simulink model "untitled"  (R2016a)
(part 5 of 5)

      mask Display: e = 0.06;c1 = [120 150 230]/255;c2 = ([120 150 230]+0)/383;c3 = ([120 150 230]+128)/383;patch([0 1 1 0],[0 0 1 1],c1);patch([0 1 1 1-e 1-e 0+e],[0 0 1 1-e 0+e 0+e],c2);patch([0 0 1 1-e 0+e 0+e],[0 1 1 1-e 1-e 0+e],c3);plot([0 1 1 0 0],[0 0 1 1 0]);disp('weights');
  "IW{2,1}(336,:)'" : Constant  Value=[0.57929667385134542;-0.78903803203994949;-0.58353476825563777;0.33313549786967889;0.5285986546184529;0.55820885952562127;-0.15831488004105437;0.041845262259330829;0.26856481467974563;0.19459032736235027]
      mask Display: e = 0.06;c1 = [120 150 230]/255;c2 = ([120 150 230]+0)/383;c3 = ([120 150 230]+128)/383;patch([0 1 1 0],[0 0 1 1],c1);patch([0 1 1 1-e 1-e 0+e],[0 0 1 1-e 0+e 0+e],c2);patch([0 0 1 1-e 0+e 0+e],[0 1 1 1-e 1-e 0+e],c3);plot([0 1 1 0 0],[0 0 1 1 0]);disp('weights');
  "IW{2,1}(337,:)'" : Constant  Value=[0.12574676902065979;0.1437303392596804;-1.0210731034248322;-0.76168646026924314;-0.43069041398995267;-0.42377470805759543;-0.92888594177016837;-0.74632505329387844;0.7159189367543517;0.21230092583291182]
      mask Display: e = 0.06;c1 = [120 150 230]/255;c2 = ([120 150 230]+0)/383;c3 = ([120 150 230]+128)/383;patch([0 1 1 0],[0 0 1 1],c1);patch([0 1 1 1-e 1-e 0+e],[0 0 1 1-e 0+e 0+e],c2);patch([0 0 1 1-e 0+e 0+e],[0 1 1 1-e 1-e 0+e],c3);plot([0 1 1 0 0],[0 0 1 1 0]);disp('weights');
  "IW{2,1}(338,:)'" : Constant  Value=[-0.87962689838467056;-0.81965574813773967;0.28812259044425648;0.6537668743923607;0.64909098817751765;0.61059084148729448;0.26188896114050575;-0.10762086270333238;-0.21705727199956715;0.37912970515334743]
      mask Display: e = 0.06;c1 = [120 150 230]/255;c2 = ([120 150 230]+0)/383;c3 = ([120 150 230]+128)/383;patch([0 1 1 0],[0 0 1 1],c1);patch([0 1 1 1-e 1-e 0+e],[0 0 1 1-e 0+e 0+e],c2);patch([0 0 1 1-e 0+e 0+e],[0 1 1 1-e 1-e 0+e],c3);plot([0 1 1 0 0],[0 0 1 1 0]);disp('weights');
  "IW{2,1}(339,:)'" : Constant  Value=[0.27086385814243769;0.13068510614586601;0.24134099648815127;-0.17928302930622905;0.82971681131724795;0.71135694066192445;-0.40450383589249345;0.42312354405169722;-0.51855680944157401;-0.31572508040730729]
      mask Display: e = 0.06;c1 = [120 150 230]/255;c2 = ([120 150 230]+0)/383;c3 = ([120 150 230]+128)/383;patch([0 1 1 0],[0 0 1 1],c1);patch([0 1 1 1-e 1-e 0+e],[0 0 1 1-e 0+e 0+e],c2);patch([0 0 1 1-e 0+e 0+e],[0 1 1 1-e 1-e 0+e],c3);plot([0 1 1 0 0],[0 0 1 1 0]);disp('weights');
  "IW{2,1}(34,:)'" : Constant  Value=[-0.0557140173148791;-0.47020898151700219;-0.10773546464442435;0.13793814800358678;0.0086097713284211119;0.054232313057208437;-1.3206898062037267;-0.5570232407889194;0.42551871848387929;-0.34291539655271253]
      mask Display: e = 0.06;c1 = [120 150 230]/255;c2 = ([120 150 230]+0)/383;c3 = ([120 150 230]+128)/383;patch([0 1 1 0],[0 0 1 1],c1);patch([0 1 1 1-e 1-e 0+e],[0 0 1 1-e 0+e 0+e],c2);patch([0 0 1 1-e 0+e 0+e],[0 1 1 1-e 1-e 0+e],c3);plot([0 1 1 0 0],[0 0 1 1 0]);disp('weights');
  "IW{2,1}(340,:)'" : Constant  Value=[0.67675704174660012;0.29451796126330321;0.96052544413959351;-0.59395989110112135;0.20754162488392677;0.042921057940714935;-0.63021749818323047;-0.10388797316770837;-0.55730109200499489;-0.8694954715348181]
      mask Display: e = 0.06;c1 = [120 150 230]/255;c2 = ([120 150 230]+0)/383;c3 = ([120 150 230]+128)/383;patch([0 1 1 0],[0 0 1 1],c1);patch([0 1 1 1-e 1-e 0+e],[0 0 1 1-e 0+e 0+e],c2);patch([0 0 1 1-e 0+e 0+e],[0 1 1 1-e 1-e 0+e],c3);plot([0 1 1 0 0],[0 0 1 1 0]);disp('weights');
  "IW{2,1}(341,:)'" : Constant  Value=[0.50441264093641003;-0.25814916788099879;0.5273849263763507;0.070525504378618736;-0.85715718129830487;0.22282102719382685;0.11137503921468966;0.15108209667316697;0.47461080777254527;-1.0033026714827977]
      mask Display: e = 0.06;c1 = [120 150 230]/255;c2 = ([120 150 230]+0)/383;c3 = ([120 150 230]+128)/383;patch([0 1 1 0],[0 0 1 1],c1);patch([0 1 1 1-e 1-e 0+e],[0 0 1 1-e 0+e 0+e],c2);patch([0 0 1 1-e 0+e 0+e],[0 1 1 1-e 1-e 0+e],c3);plot([0 1 1 0 0],[0 0 1 1 0]);disp('weights');
  "IW{2,1}(342,:)'" : Constant  Value=[-0.87120151971974302;-0.21701047633843468;0.22343161213378757;-0.6224636306634812;-0.18118189058358763;0.77302593300289923;0.063648446964245042;-0.33024680040415128;0.61297869563987939;0.62661425915964464]
      mask Display: e = 0.06;c1 = [120 150 230]/255;c2 = ([120 150 230]+0)/383;c3 = ([120 150 230]+128)/383;patch([0 1 1 0],[0 0 1 1],c1);patch([0 1 1 1-e 1-e 0+e],[0 0 1 1-e 0+e 0+e],c2);patch([0 0 1 1-e 0+e 0+e],[0 1 1 1-e 1-e 0+e],c3);plot([0 1 1 0 0],[0 0 1 1 0]);disp('weights');
  "IW{2,1}(343,:)'" : Constant  Value=[0.54778667415285753;0.58942993005933753;-0.82715214046328522;-0.42267861457146078;1.217645261929982;0.41030733543075537;-0.48105634702976574;-0.63559529927366576;0.44469140820414194;0.68942657577069366]
      mask Display: e = 0.06;c1 = [120 150 230]/255;c2 = ([120 150 230]+0)/383;c3 = ([120 150 230]+128)/383;patch([0 1 1 0],[0 0 1 1],c1);patch([0 1 1 1-e 1-e 0+e],[0 0 1 1-e 0+e 0+e],c2);patch([0 0 1 1-e 0+e 0+e],[0 1 1 1-e 1-e 0+e],c3);plot([0 1 1 0 0],[0 0 1 1 0]);disp('weights');
  "IW{2,1}(344,:)'" : Constant  Value=[0.80938005282717895;0.85758702347541127;0.3249857359421256;0.068660961528306613;-0.48979054333668026;0.68731063432055062;0.13924348683501817;0.12645778251410511;0.42804861718142606;0.30521647390760931]
      mask Display: e = 0.06;c1 = [120 150 230]/255;c2 = ([120 150 230]+0)/383;c3 = ([120 150 230]+128)/383;patch([0 1 1 0],[0 0 1 1],c1);patch([0 1 1 1-e 1-e 0+e],[0 0 1 1-e 0+e 0+e],c2);patch([0 0 1 1-e 0+e 0+e],[0 1 1 1-e 1-e 0+e],c3);plot([0 1 1 0 0],[0 0 1 1 0]);disp('weights');
  "IW{2,1}(345,:)'" : Constant  Value=[-0.40642866004188194;0.024144431082813451;-1.0230073088457663;-0.95248385746212494;0.72926259142932381;0.30665424718799306;-0.96967684388735786;-0.20945754302261479;-0.39772236198321215;0.71881238198133679]
      mask Display: e = 0.06;c1 = [120 150 230]/255;c2 = ([120 150 230]+0)/383;c3 = ([120 150 230]+128)/383;patch([0 1 1 0],[0 0 1 1],c1);patch([0 1 1 1-e 1-e 0+e],[0 0 1 1-e 0+e 0+e],c2);patch([0 0 1 1-e 0+e 0+e],[0 1 1 1-e 1-e 0+e],c3);plot([0 1 1 0 0],[0 0 1 1 0]);disp('weights');
  "IW{2,1}(346,:)'" : Constant  Value=[1.3740864718913919;0.22871612043931461;-0.044941575484340718;0.6616130294723428;-0.2189939835849456;0.57109137173194335;-0.48540204603619996;0.37566365540689645;-0.52135066902196248;0.10168152866206817]
      mask Display: e = 0.06;c1 = [120 150 230]/255;c2 = ([120 150 230]+0)/383;c3 = ([120 150 230]+128)/383;patch([0 1 1 0],[0 0 1 1],c1);patch([0 1 1 1-e 1-e 0+e],[0 0 1 1-e 0+e 0+e],c2);patch([0 0 1 1-e 0+e 0+e],[0 1 1 1-e 1-e 0+e],c3);plot([0 1 1 0 0],[0 0 1 1 0]);disp('weights');
  "IW{2,1}(347,:)'" : Constant  Value=[0.29248266901944847;-0.33621530376745251;-0.036164134244412352;-0.014456472781074908;-0.29890516910801945;-0.0024103397765527501;-1.0913384164665245;-0.58722890720668386;0.20481619829248193;0.040425924896277027]
      mask Display: e = 0.06;c1 = [120 150 230]/255;c2 = ([120 150 230]+0)/383;c3 = ([120 150 230]+128)/383;patch([0 1 1 0],[0 0 1 1],c1);patch([0 1 1 1-e 1-e 0+e],[0 0 1 1-e 0+e 0+e],c2);patch([0 0 1 1-e 0+e 0+e],[0 1 1 1-e 1-e 0+e],c3);plot([0 1 1 0 0],[0 0 1 1 0]);disp('weights');
  "IW{2,1}(348,:)'" : Constant  Value=[0.066871656522572154;-0.82037360738171827;-1.1829225017254741;-0.11652694921625323;0.4760845225460491;-0.24870797400433475;-0.33779280137749595;-0.3870624604689627;1.1401042150744649;-0.12733608401848256]
      mask Display: e = 0.06;c1 = [120 150 230]/255;c2 = ([120 150 230]+0)/383;c3 = ([120 150 230]+128)/383;patch([0 1 1 0],[0 0 1 1],c1);patch([0 1 1 1-e 1-e 0+e],[0 0 1 1-e 0+e 0+e],c2);patch([0 0 1 1-e 0+e 0+e],[0 1 1 1-e 1-e 0+e],c3);plot([0 1 1 0 0],[0 0 1 1 0]);disp('weights');
  "IW{2,1}(349,:)'" : Constant  Value=[-0.56516748165346065;0.60421432434592071;0.21477667628823882;-0.37962152691604534;0.054230828961916944;0.97713641951169294;0.34032689677335731;-0.22209678073966532;0.69491764586228777;0.40837973620708379]
      mask Display: e = 0.06;c1 = [120 150 230]/255;c2 = ([120 150 230]+0)/383;c3 = ([120 150 230]+128)/383;patch([0 1 1 0],[0 0 1 1],c1);patch([0 1 1 1-e 1-e 0+e],[0 0 1 1-e 0+e 0+e],c2);patch([0 0 1 1-e 0+e 0+e],[0 1 1 1-e 1-e 0+e],c3);plot([0 1 1 0 0],[0 0 1 1 0]);disp('weights');
  "IW{2,1}(35,:)'" : Constant  Value=[-0.25760074676464095;-0.28380985445048007;0.43164066332849033;0.23220168279956635;0.56055874690034724;0.81979353327154014;0.072753955941441018;-0.014426558695554342;-0.071318431922984982;-0.47703848064843912]
      mask Display: e = 0.06;c1 = [120 150 230]/255;c2 = ([120 150 230]+0)/383;c3 = ([120 150 230]+128)/383;patch([0 1 1 0],[0 0 1 1],c1);patch([0 1 1 1-e 1-e 0+e],[0 0 1 1-e 0+e 0+e],c2);patch([0 0 1 1-e 0+e 0+e],[0 1 1 1-e 1-e 0+e],c3);plot([0 1 1 0 0],[0 0 1 1 0]);disp('weights');
  "IW{2,1}(350,:)'" : Constant  Value=[0.051988509795972401;-0.013574912572032562;-0.28560378849152268;-0.32799987653965129;1.3044047508544199;0.43736308271531554;0.071266929416620328;0.73520543165915775;0.10884565625748632;0.25695621700303634]
      mask Display: e = 0.06;c1 = [120 150 230]/255;c2 = ([120 150 230]+0)/383;c3 = ([120 150 230]+128)/383;patch([0 1 1 0],[0 0 1 1],c1);patch([0 1 1 1-e 1-e 0+e],[0 0 1 1-e 0+e 0+e],c2);patch([0 0 1 1-e 0+e 0+e],[0 1 1 1-e 1-e 0+e],c3);plot([0 1 1 0 0],[0 0 1 1 0]);disp('weights');
  "IW{2,1}(351,:)'" : Constant  Value=[0.4568469818767768;0.33566359392055301;0.5049775876308441;-1.1445276549307513;-0.062160417784633715;0.36349307929056063;0.056913164235412275;0.10142049361460195;0.83007833319535318;-0.92565819038237251]
      mask Display: e = 0.06;c1 = [120 150 230]/255;c2 = ([120 150 230]+0)/383;c3 = ([120 150 230]+128)/383;patch([0 1 1 0],[0 0 1 1],c1);patch([0 1 1 1-e 1-e 0+e],[0 0 1 1-e 0+e 0+e],c2);patch([0 0 1 1-e 0+e 0+e],[0 1 1 1-e 1-e 0+e],c3);plot([0 1 1 0 0],[0 0 1 1 0]);disp('weights');
  "IW{2,1}(352,:)'" : Constant  Value=[-0.88703160304489614;-0.95132318021638718;-0.071861533145697376;-0.42033187199910793;-0.68579336170567229;0.35422349162839978;-0.20304709238721164;-0.13214983308353762;0.47337758454097267;0.15078308159578074]
      mask Display: e = 0.06;c1 = [120 150 230]/255;c2 = ([120 150 230]+0)/383;c3 = ([120 150 230]+128)/383;patch([0 1 1 0],[0 0 1 1],c1);patch([0 1 1 1-e 1-e 0+e],[0 0 1 1-e 0+e 0+e],c2);patch([0 0 1 1-e 0+e 0+e],[0 1 1 1-e 1-e 0+e],c3);plot([0 1 1 0 0],[0 0 1 1 0]);disp('weights');
  "IW{2,1}(353,:)'" : Constant  Value=[0.53782537655597384;-1.0045125582834515;0.30134495879826806;0.54230596767481742;-0.11476579937739612;-0.31631782729707281;-0.49763177218689092;0.47994082141207151;-0.026801952215077307;0.25824481163233315]
      mask Display: e = 0.06;c1 = [120 150 230]/255;c2 = ([120 150 230]+0)/383;c3 = ([120 150 230]+128)/383;patch([0 1 1 0],[0 0 1 1],c1);patch([0 1 1 1-e 1-e 0+e],[0 0 1 1-e 0+e 0+e],c2);patch([0 0 1 1-e 0+e 0+e],[0 1 1 1-e 1-e 0+e],c3);plot([0 1 1 0 0],[0 0 1 1 0]);disp('weights');
  "IW{2,1}(354,:)'" : Constant  Value=[-0.41358424712483965;-0.4329293804487403;-0.029573647317088669;-1.2035042893054049;-0.52506569755795507;-0.090459746021540999;-0.83104269463153191;-0.56242756805362537;0.80415249041968218;-0.76295105731743029]
      mask Display: e = 0.06;c1 = [120 150 230]/255;c2 = ([120 150 230]+0)/383;c3 = ([120 150 230]+128)/383;patch([0 1 1 0],[0 0 1 1],c1);patch([0 1 1 1-e 1-e 0+e],[0 0 1 1-e 0+e 0+e],c2);patch([0 0 1 1-e 0+e 0+e],[0 1 1 1-e 1-e 0+e],c3);plot([0 1 1 0 0],[0 0 1 1 0]);disp('weights');
  "IW{2,1}(355,:)'" : Constant  Value=[0.26135712427590718;0.32178024612794087;-0.2015877707363507;-0.56893396997562329;0.85311359616962334;0.77329604180705036;0.18423955850823046;-0.22726419478735588;1.0460001041156679;-1.1010704916311156]
      mask Display: e = 0.06;c1 = [120 150 230]/255;c2 = ([120 150 230]+0)/383;c3 = ([120 150 230]+128)/383;patch([0 1 1 0],[0 0 1 1],c1);patch([0 1 1 1-e 1-e 0+e],[0 0 1 1-e 0+e 0+e],c2);patch([0 0 1 1-e 0+e 0+e],[0 1 1 1-e 1-e 0+e],c3);plot([0 1 1 0 0],[0 0 1 1 0]);disp('weights');
  "IW{2,1}(356,:)'" : Constant  Value=[0.12593724696620373;-0.88317548884339514;0.61782360547129;0.3650623555503672;0.84964646887594097;-0.060897734797931147;-0.09226266712536807;0.95533325883592723;0.21782434532452424;-0.5450519926170927]
      mask Display: e = 0.06;c1 = [120 150 230]/255;c2 = ([120 150 230]+0)/383;c3 = ([120 150 230]+128)/383;patch([0 1 1 0],[0 0 1 1],c1);patch([0 1 1 1-e 1-e 0+e],[0 0 1 1-e 0+e 0+e],c2);patch([0 0 1 1-e 0+e 0+e],[0 1 1 1-e 1-e 0+e],c3);plot([0 1 1 0 0],[0 0 1 1 0]);disp('weights');
  "IW{2,1}(357,:)'" : Constant  Value=[1.2836518532371932;0.096160776666661396;0.21514725496260828;-0.14993645779627218;0.77032281988344842;-0.088545879174764419;0.080372411198171567;0.27039995283895241;0.13932491029297017;-1.1624821130974141]
      mask Display: e = 0.06;c1 = [120 150 230]/255;c2 = ([120 150 230]+0)/383;c3 = ([120 150 230]+128)/383;patch([0 1 1 0],[0 0 1 1],c1);patch([0 1 1 1-e 1-e 0+e],[0 0 1 1-e 0+e 0+e],c2);patch([0 0 1 1-e 0+e 0+e],[0 1 1 1-e 1-e 0+e],c3);plot([0 1 1 0 0],[0 0 1 1 0]);disp('weights');
  "IW{2,1}(358,:)'" : Constant  Value=[0.41363822429458708;-0.50795929263917061;-1.0166610274774324;0.17985534655157204;0.59634524812206458;-0.1370381387001669;-0.95345344550304645;-0.40283143884480399;-0.10361796483681018;-0.34231456711728475]
      mask Display: e = 0.06;c1 = [120 150 230]/255;c2 = ([120 150 230]+0)/383;c3 = ([120 150 230]+128)/383;patch([0 1 1 0],[0 0 1 1],c1);patch([0 1 1 1-e 1-e 0+e],[0 0 1 1-e 0+e 0+e],c2);patch([0 0 1 1-e 0+e 0+e],[0 1 1 1-e 1-e 0+e],c3);plot([0 1 1 0 0],[0 0 1 1 0]);disp('weights');
  "IW{2,1}(359,:)'" : Constant  Value=[0.4130436215767474;-0.183058653765241;0.33510684212361275;0.32830599576756209;0.47422521040876997;0.14706087537797086;-0.8502254133587428;0.51550316311474309;-0.52704969245761002;-1.083761279133916]
      mask Display: e = 0.06;c1 = [120 150 230]/255;c2 = ([120 150 230]+0)/383;c3 = ([120 150 230]+128)/383;patch([0 1 1 0],[0 0 1 1],c1);patch([0 1 1 1-e 1-e 0+e],[0 0 1 1-e 0+e 0+e],c2);patch([0 0 1 1-e 0+e 0+e],[0 1 1 1-e 1-e 0+e],c3);plot([0 1 1 0 0],[0 0 1 1 0]);disp('weights');
  "IW{2,1}(36,:)'" : Constant  Value=[-0.66982395148976859;-0.81608991183897839;0.86201861625844423;-0.088516333606687314;-0.73434972184789205;0.38474377958596861;0.013093561446158308;-0.33585323345285761;0.32605230677276575;-0.28115912300023482]
      mask Display: e = 0.06;c1 = [120 150 230]/255;c2 = ([120 150 230]+0)/383;c3 = ([120 150 230]+128)/383;patch([0 1 1 0],[0 0 1 1],c1);patch([0 1 1 1-e 1-e 0+e],[0 0 1 1-e 0+e 0+e],c2);patch([0 0 1 1-e 0+e 0+e],[0 1 1 1-e 1-e 0+e],c3);plot([0 1 1 0 0],[0 0 1 1 0]);disp('weights');
  "IW{2,1}(360,:)'" : Constant  Value=[0.52438688001317146;0.59324965310100786;-0.52664342692991439;-0.5071792695022479;-0.35564302439400591;0.41090017775667498;-0.94384701830625062;-0.78061911572039744;0.89594149401490297;-0.098471901579605281]
      mask Display: e = 0.06;c1 = [120 150 230]/255;c2 = ([120 150 230]+0)/383;c3 = ([120 150 230]+128)/383;patch([0 1 1 0],[0 0 1 1],c1);patch([0 1 1 1-e 1-e 0+e],[0 0 1 1-e 0+e 0+e],c2);patch([0 0 1 1-e 0+e 0+e],[0 1 1 1-e 1-e 0+e],c3);plot([0 1 1 0 0],[0 0 1 1 0]);disp('weights');
  "IW{2,1}(361,:)'" : Constant  Value=[0.70715762696726192;-0.29748621851513668;-0.78388707278358016;0.18203663042024709;-0.54727256061737262;-0.31606523699953892;-0.73697892746355853;-0.69113299453781996;0.86296120234346929;-0.022153904020826731]
      mask Display: e = 0.06;c1 = [120 150 230]/255;c2 = ([120 150 230]+0)/383;c3 = ([120 150 230]+128)/383;patch([0 1 1 0],[0 0 1 1],c1);patch([0 1 1 1-e 1-e 0+e],[0 0 1 1-e 0+e 0+e],c2);patch([0 0 1 1-e 0+e 0+e],[0 1 1 1-e 1-e 0+e],c3);plot([0 1 1 0 0],[0 0 1 1 0]);disp('weights');
  "IW{2,1}(362,:)'" : Constant  Value=[-0.37733059061743363;-0.95244251436414906;-0.08604930474107389;-0.33510485443863969;0.89280504182612863;0.17645970421334201;-0.57215399989368076;-0.4509902143881282;0.49780293873215242;-1.0224805512993878]
      mask Display: e = 0.06;c1 = [120 150 230]/255;c2 = ([120 150 230]+0)/383;c3 = ([120 150 230]+128)/383;patch([0 1 1 0],[0 0 1 1],c1);patch([0 1 1 1-e 1-e 0+e],[0 0 1 1-e 0+e 0+e],c2);patch([0 0 1 1-e 0+e 0+e],[0 1 1 1-e 1-e 0+e],c3);plot([0 1 1 0 0],[0 0 1 1 0]);disp('weights');
  "IW{2,1}(363,:)'" : Constant  Value=[-0.56080354128068299;-1.0605260184533114;0.35981638767902596;0.67836990066402381;-0.15829977938426784;0.53115719541767592;0.041016715425137185;0.36011837247641632;0.033180891712814242;0.44906526055357837]
      mask Display: e = 0.06;c1 = [120 150 230]/255;c2 = ([120 150 230]+0)/383;c3 = ([120 150 230]+128)/383;patch([0 1 1 0],[0 0 1 1],c1);patch([0 1 1 1-e 1-e 0+e],[0 0 1 1-e 0+e 0+e],c2);patch([0 0 1 1-e 0+e 0+e],[0 1 1 1-e 1-e 0+e],c3);plot([0 1 1 0 0],[0 0 1 1 0]);disp('weights');
  "IW{2,1}(364,:)'" : Constant  Value=[-0.31815206379702421;-0.82038866221530804;0.25142504723102077;-0.026051677533059425;0.34283223282559894;0.73415671366936519;0.16861767882705381;0.26155466351752144;0.44510737053685528;-0.90398222557634356]
      mask Display: e = 0.06;c1 = [120 150 230]/255;c2 = ([120 150 230]+0)/383;c3 = ([120 150 230]+128)/383;patch([0 1 1 0],[0 0 1 1],c1);patch([0 1 1 1-e 1-e 0+e],[0 0 1 1-e 0+e 0+e],c2);patch([0 0 1 1-e 0+e 0+e],[0 1 1 1-e 1-e 0+e],c3);plot([0 1 1 0 0],[0 0 1 1 0]);disp('weights');
  "IW{2,1}(365,:)'" : Constant  Value=[1.0062343251038501;0.12160712684179426;-0.91758803753298757;-0.049457295597564344;0.15850694661352183;0.35359237912571306;0.51010609936155371;-0.30175649394852433;1.0850776063772001;0.23361164639195278]
      mask Display: e = 0.06;c1 = [120 150 230]/255;c2 = ([120 150 230]+0)/383;c3 = ([120 150 230]+128)/383;patch([0 1 1 0],[0 0 1 1],c1);patch([0 1 1 1-e 1-e 0+e],[0 0 1 1-e 0+e 0+e],c2);patch([0 0 1 1-e 0+e 0+e],[0 1 1 1-e 1-e 0+e],c3);plot([0 1 1 0 0],[0 0 1 1 0]);disp('weights');
  "IW{2,1}(366,:)'" : Constant  Value=[-0.2240900931176289;-0.28331587690497984;-0.033168202063454083;-0.47831796955342859;0.37256137876802758;0.85409870847040037;0.61399183709175498;-0.45276395856936563;0.75978964299335527;0.25665226409514563]
      mask Display: e = 0.06;c1 = [120 150 230]/255;c2 = ([120 150 230]+0)/383;c3 = ([120 150 230]+128)/383;patch([0 1 1 0],[0 0 1 1],c1);patch([0 1 1 1-e 1-e 0+e],[0 0 1 1-e 0+e 0+e],c2);patch([0 0 1 1-e 0+e 0+e],[0 1 1 1-e 1-e 0+e],c3);plot([0 1 1 0 0],[0 0 1 1 0]);disp('weights');
  "IW{2,1}(367,:)'" : Constant  Value=[-0.45202183027849552;-0.67413360670780687;0.43829045446701459;0.33436250889631647;-0.43135954889503847;0.7566209115469279;0.35700045752867021;-0.0073657033657865967;-0.30937113260961435;0.15982677870068024]
      mask Display: e = 0.06;c1 = [120 150 230]/255;c2 = ([120 150 230]+0)/383;c3 = ([120 150 230]+128)/383;patch([0 1 1 0],[0 0 1 1],c1);patch([0 1 1 1-e 1-e 0+e],[0 0 1 1-e 0+e 0+e],c2);patch([0 0 1 1-e 0+e 0+e],[0 1 1 1-e 1-e 0+e],c3);plot([0 1 1 0 0],[0 0 1 1 0]);disp('weights');
  "IW{2,1}(368,:)'" : Constant  Value=[0.95528875264789559;0.048810392853254642;-0.15128752608298668;0.032095412547711061;-0.31225439409768863;0.25663734424455348;-0.61248754250215831;0.30115089168303327;-0.27071473827486647;0.94323215038612196]
      mask Display: e = 0.06;c1 = [120 150 230]/255;c2 = ([120 150 230]+0)/383;c3 = ([120 150 230]+128)/383;patch([0 1 1 0],[0 0 1 1],c1);patch([0 1 1 1-e 1-e 0+e],[0 0 1 1-e 0+e 0+e],c2);patch([0 0 1 1-e 0+e 0+e],[0 1 1 1-e 1-e 0+e],c3);plot([0 1 1 0 0],[0 0 1 1 0]);disp('weights');
  "IW{2,1}(369,:)'" : Constant  Value=[-0.051310532937357101;-0.1123729590216242;-0.1011144072681802;-0.75279123224713984;0.37434102186839463;0.75956087229758518;0.096032414864186733;-0.61036293648674522;0.45034131445111431;-0.34934417014295077]
      mask Display: e = 0.06;c1 = [120 150 230]/255;c2 = ([120 150 230]+0)/383;c3 = ([120 150 230]+128)/383;patch([0 1 1 0],[0 0 1 1],c1);patch([0 1 1 1-e 1-e 0+e],[0 0 1 1-e 0+e 0+e],c2);patch([0 0 1 1-e 0+e 0+e],[0 1 1 1-e 1-e 0+e],c3);plot([0 1 1 0 0],[0 0 1 1 0]);disp('weights');
  "IW{2,1}(37,:)'" : Constant  Value=[-0.45346601004557541;-0.92638798216420537;-0.0036014599512361883;-0.79717972863810749;0.79441797608476394;-0.04420198991017954;-0.35129188467774886;-0.12314527532235071;-0.23667445475210086;-0.26552873426458157]
      mask Display: e = 0.06;c1 = [120 150 230]/255;c2 = ([120 150 230]+0)/383;c3 = ([120 150 230]+128)/383;patch([0 1 1 0],[0 0 1 1],c1);patch([0 1 1 1-e 1-e 0+e],[0 0 1 1-e 0+e 0+e],c2);patch([0 0 1 1-e 0+e 0+e],[0 1 1 1-e 1-e 0+e],c3);plot([0 1 1 0 0],[0 0 1 1 0]);disp('weights');
  "IW{2,1}(370,:)'" : Constant  Value=[0.59495595976997395;-0.59092895941974555;-0.088906223996489786;0.35401334649079008;0.87623876698045877;0.5923361038192041;-0.67965672068874228;-0.63546176058554171;-0.38542351378121636;-0.12205619773779863]
      mask Display: e = 0.06;c1 = [120 150 230]/255;c2 = ([120 150 230]+0)/383;c3 = ([120 150 230]+128)/383;patch([0 1 1 0],[0 0 1 1],c1);patch([0 1 1 1-e 1-e 0+e],[0 0 1 1-e 0+e 0+e],c2);patch([0 0 1 1-e 0+e 0+e],[0 1 1 1-e 1-e 0+e],c3);plot([0 1 1 0 0],[0 0 1 1 0]);disp('weights');
  "IW{2,1}(371,:)'" : Constant  Value=[0.23627638669211504;-0.28592154184872304;-0.29692503487187927;-0.99950292154989961;-0.10979879275554638;0.16581367426394772;0.4051848883087244;0.44661122338547038;1.1527488770938223;-0.8003466806299766]
      mask Display: e = 0.06;c1 = [120 150 230]/255;c2 = ([120 150 230]+0)/383;c3 = ([120 150 230]+128)/383;patch([0 1 1 0],[0 0 1 1],c1);patch([0 1 1 1-e 1-e 0+e],[0 0 1 1-e 0+e 0+e],c2);patch([0 0 1 1-e 0+e 0+e],[0 1 1 1-e 1-e 0+e],c3);plot([0 1 1 0 0],[0 0 1 1 0]);disp('weights');
  "IW{2,1}(372,:)'" : Constant  Value=[-0.67098048884064265;-0.98252043663715161;-0.3920559632902213;0.779961268050263;0.77809817028453743;0.83806676396730717;-0.3801704597740615;-0.49630685958044063;0.23963829386122235;0.46454961442588549]
      mask Display: e = 0.06;c1 = [120 150 230]/255;c2 = ([120 150 230]+0)/383;c3 = ([120 150 230]+128)/383;patch([0 1 1 0],[0 0 1 1],c1);patch([0 1 1 1-e 1-e 0+e],[0 0 1 1-e 0+e 0+e],c2);patch([0 0 1 1-e 0+e 0+e],[0 1 1 1-e 1-e 0+e],c3);plot([0 1 1 0 0],[0 0 1 1 0]);disp('weights');
  "IW{2,1}(373,:)'" : Constant  Value=[-0.49454221335119214;-1.0450847269589292;-1.2131601353640342;0.19065975541700025;0.9158867788925914;0.6939355543607878;-0.23992063893135473;-0.043254272936928427;0.53344248088877999;0.36266718936114972]
      mask Display: e = 0.06;c1 = [120 150 230]/255;c2 = ([120 150 230]+0)/383;c3 = ([120 150 230]+128)/383;patch([0 1 1 0],[0 0 1 1],c1);patch([0 1 1 1-e 1-e 0+e],[0 0 1 1-e 0+e 0+e],c2);patch([0 0 1 1-e 0+e 0+e],[0 1 1 1-e 1-e 0+e],c3);plot([0 1 1 0 0],[0 0 1 1 0]);disp('weights');
  "IW{2,1}(374,:)'" : Constant  Value=[0.52831252828886033;0.49789404044819491;-0.56854297226354911;-0.28551257859276452;1.058182111640938;0.20169785458295797;-0.79337331277396761;-0.20030943205965893;0.22429760134665144;0.35081341786804915]
      mask Display: e = 0.06;c1 = [120 150 230]/255;c2 = ([120 150 230]+0)/383;c3 = ([120 150 230]+128)/383;patch([0 1 1 0],[0 0 1 1],c1);patch([0 1 1 1-e 1-e 0+e],[0 0 1 1-e 0+e 0+e],c2);patch([0 0 1 1-e 0+e 0+e],[0 1 1 1-e 1-e 0+e],c3);plot([0 1 1 0 0],[0 0 1 1 0]);disp('weights');
  "IW{2,1}(375,:)'" : Constant  Value=[0.17165827901943526;-0.59807532697402133;-0.23461538714994559;0.3620802632515544;0.58865111309730611;0.48827830971295988;-0.81328901714558399;-0.20994398652083701;-0.2557698826205827;-0.68153095140306563]
      mask Display: e = 0.06;c1 = [120 150 230]/255;c2 = ([120 150 230]+0)/383;c3 = ([120 150 230]+128)/383;patch([0 1 1 0],[0 0 1 1],c1);patch([0 1 1 1-e 1-e 0+e],[0 0 1 1-e 0+e 0+e],c2);patch([0 0 1 1-e 0+e 0+e],[0 1 1 1-e 1-e 0+e],c3);plot([0 1 1 0 0],[0 0 1 1 0]);disp('weights');
  "IW{2,1}(376,:)'" : Constant  Value=[0.18882072426149238;-0.96039315601962194;-0.64055183679610284;-0.0022176093312210876;-0.20906800651172366;-0.083330630773641667;-0.60407417176194278;0.30773624057581178;0.75392831287590067;-0.33283636993213683]
      mask Display: e = 0.06;c1 = [120 150 230]/255;c2 = ([120 150 230]+0)/383;c3 = ([120 150 230]+128)/383;patch([0 1 1 0],[0 0 1 1],c1);patch([0 1 1 1-e 1-e 0+e],[0 0 1 1-e 0+e 0+e],c2);patch([0 0 1 1-e 0+e 0+e],[0 1 1 1-e 1-e 0+e],c3);plot([0 1 1 0 0],[0 0 1 1 0]);disp('weights');
  "IW{2,1}(377,:)'" : Constant  Value=[0.91883596669132717;0.42015327502381139;-0.30809105806961579;-0.62091835192639822;1.3161283216594084;0.1123718750814523;0.23275746837669942;0.1431287770758021;-0.32232411769425245;0.019804204996174857]
      mask Display: e = 0.06;c1 = [120 150 230]/255;c2 = ([120 150 230]+0)/383;c3 = ([120 150 230]+128)/383;patch([0 1 1 0],[0 0 1 1],c1);patch([0 1 1 1-e 1-e 0+e],[0 0 1 1-e 0+e 0+e],c2);patch([0 0 1 1-e 0+e 0+e],[0 1 1 1-e 1-e 0+e],c3);plot([0 1 1 0 0],[0 0 1 1 0]);disp('weights');
  "IW{2,1}(378,:)'" : Constant  Value=[0.5825692951649375;0.70083457158090212;0.25126594258432811;-0.14290908254612986;0.98323841541436563;0.82148192814072551;0.30653741293257231;0.32637465094842305;-0.42557648522958469;-0.1071596049987209]
      mask Display: e = 0.06;c1 = [120 150 230]/255;c2 = ([120 150 230]+0)/383;c3 = ([120 150 230]+128)/383;patch([0 1 1 0],[0 0 1 1],c1);patch([0 1 1 1-e 1-e 0+e],[0 0 1 1-e 0+e 0+e],c2);patch([0 0 1 1-e 0+e 0+e],[0 1 1 1-e 1-e 0+e],c3);plot([0 1 1 0 0],[0 0 1 1 0]);disp('weights');
  "IW{2,1}(379,:)'" : Constant  Value=[0.067873117132048827;0.34066692543185034;-0.83071286589236282;-1.1852621184232368;0.99534514041640643;0.65449496890547243;0.4920908950069216;0.17363323899811353;0.95463083668841919;-0.68593034199389435]
      mask Display: e = 0.06;c1 = [120 150 230]/255;c2 = ([120 150 230]+0)/383;c3 = ([120 150 230]+128)/383;patch([0 1 1 0],[0 0 1 1],c1);patch([0 1 1 1-e 1-e 0+e],[0 0 1 1-e 0+e 0+e],c2);patch([0 0 1 1-e 0+e 0+e],[0 1 1 1-e 1-e 0+e],c3);plot([0 1 1 0 0],[0 0 1 1 0]);disp('weights');
  "IW{2,1}(38,:)'" : Constant  Value=[1.0176454852874275;-0.57110172777058854;-0.10154038575350374;-0.12130944587593001;-0.61723935296532928;-0.50769180359267652;-0.94794463319835709;0.36589623727227233;-0.15209055037516442;-0.50866293296671894]
      mask Display: e = 0.06;c1 = [120 150 230]/255;c2 = ([120 150 230]+0)/383;c3 = ([120 150 230]+128)/383;patch([0 1 1 0],[0 0 1 1],c1);patch([0 1 1 1-e 1-e 0+e],[0 0 1 1-e 0+e 0+e],c2);patch([0 0 1 1-e 0+e 0+e],[0 1 1 1-e 1-e 0+e],c3);plot([0 1 1 0 0],[0 0 1 1 0]);disp('weights');
  "IW{2,1}(380,:)'" : Constant  Value=[0.39027438812921411;0.11135155986026858;0.082198015437587979;0.44973579359541666;0.91763084545441942;0.54456614319151475;-0.4839503194867722;0.15522017542824901;0.45906791664851093;0.08571483195668822]
      mask Display: e = 0.06;c1 = [120 150 230]/255;c2 = ([120 150 230]+0)/383;c3 = ([120 150 230]+128)/383;patch([0 1 1 0],[0 0 1 1],c1);patch([0 1 1 1-e 1-e 0+e],[0 0 1 1-e 0+e 0+e],c2);patch([0 0 1 1-e 0+e 0+e],[0 1 1 1-e 1-e 0+e],c3);plot([0 1 1 0 0],[0 0 1 1 0]);disp('weights');
  "IW{2,1}(381,:)'" : Constant  Value=[0.23634239449334549;-1.1454852690497903;-0.43822619213562503;0.30874423996541078;0.15152142259814372;-0.24824610051058582;-1.0155078329131138;-0.24224985546413297;-0.11378539952647845;-0.3272967417033017]
      mask Display: e = 0.06;c1 = [120 150 230]/255;c2 = ([120 150 230]+0)/383;c3 = ([120 150 230]+128)/383;patch([0 1 1 0],[0 0 1 1],c1);patch([0 1 1 1-e 1-e 0+e],[0 0 1 1-e 0+e 0+e],c2);patch([0 0 1 1-e 0+e 0+e],[0 1 1 1-e 1-e 0+e],c3);plot([0 1 1 0 0],[0 0 1 1 0]);disp('weights');
  "IW{2,1}(382,:)'" : Constant  Value=[-0.22991551162271467;-0.63862199556114141;-0.67726567141322258;-0.23729095792837873;0.99088879738604818;-0.0075835736697616452;-0.9510440356087293;-0.70277866816937662;0.70065629790162243;0.67077855946559384]
      mask Display: e = 0.06;c1 = [120 150 230]/255;c2 = ([120 150 230]+0)/383;c3 = ([120 150 230]+128)/383;patch([0 1 1 0],[0 0 1 1],c1);patch([0 1 1 1-e 1-e 0+e],[0 0 1 1-e 0+e 0+e],c2);patch([0 0 1 1-e 0+e 0+e],[0 1 1 1-e 1-e 0+e],c3);plot([0 1 1 0 0],[0 0 1 1 0]);disp('weights');
  "IW{2,1}(383,:)'" : Constant  Value=[0.029377421308622795;0.081865793648851784;0.1586978216423881;-0.37283036002059583;1.0733114765097016;0.77945983011711917;-0.29490006630719112;-0.083644275526950571;0.50738212120290205;-0.77412461866613413]
      mask Display: e = 0.06;c1 = [120 150 230]/255;c2 = ([120 150 230]+0)/383;c3 = ([120 150 230]+128)/383;patch([0 1 1 0],[0 0 1 1],c1);patch([0 1 1 1-e 1-e 0+e],[0 0 1 1-e 0+e 0+e],c2);patch([0 0 1 1-e 0+e 0+e],[0 1 1 1-e 1-e 0+e],c3);plot([0 1 1 0 0],[0 0 1 1 0]);disp('weights');
  "IW{2,1}(384,:)'" : Constant  Value=[0.77150019696560301;-0.40932595673152827;-1.0212764745504839;0.31998851121365385;-0.8703097705994336;0.15381272100057128;0.24227169198621826;-0.50335287202275203;0.89470534145456782;0.60819214328980975]
      mask Display: e = 0.06;c1 = [120 150 230]/255;c2 = ([120 150 230]+0)/383;c3 = ([120 150 230]+128)/383;patch([0 1 1 0],[0 0 1 1],c1);patch([0 1 1 1-e 1-e 0+e],[0 0 1 1-e 0+e 0+e],c2);patch([0 0 1 1-e 0+e 0+e],[0 1 1 1-e 1-e 0+e],c3);plot([0 1 1 0 0],[0 0 1 1 0]);disp('weights');
  "IW{2,1}(385,:)'" : Constant  Value=[0.48074217131819841;-0.081429211709729804;0.71738745071773391;-0.47073209327802656;0.85252978010148128;0.31260802639993129;0.31906243004122881;0.52542024434062928;0.4607345761953372;0.65626975846787738]
      mask Display: e = 0.06;c1 = [120 150 230]/255;c2 = ([120 150 230]+0)/383;c3 = ([120 150 230]+128)/383;patch([0 1 1 0],[0 0 1 1],c1);patch([0 1 1 1-e 1-e 0+e],[0 0 1 1-e 0+e 0+e],c2);patch([0 0 1 1-e 0+e 0+e],[0 1 1 1-e 1-e 0+e],c3);plot([0 1 1 0 0],[0 0 1 1 0]);disp('weights');
  "IW{2,1}(386,:)'" : Constant  Value=[0.9773101786102919;0.38895653645806255;-0.082990946909231089;0.48058795843869551;0.36991702220931233;0.12152972258872163;-0.34875372190853987;-0.23128180331648562;0.77862970656961372;-0.70491560167381651]
      mask Display: e = 0.06;c1 = [120 150 230]/255;c2 = ([120 150 230]+0)/383;c3 = ([120 150 230]+128)/383;patch([0 1 1 0],[0 0 1 1],c1);patch([0 1 1 1-e 1-e 0+e],[0 0 1 1-e 0+e 0+e],c2);patch([0 0 1 1-e 0+e 0+e],[0 1 1 1-e 1-e 0+e],c3);plot([0 1 1 0 0],[0 0 1 1 0]);disp('weights');
  "IW{2,1}(387,:)'" : Constant  Value=[-0.1799774944321787;-0.75122758868235873;0.42409351106862148;0.061085281745235913;0.57526239898938214;0.0011256081687973651;-0.85118398083550062;0.59688394425738656;-0.49207775182758517;-0.062698348134811177]
      mask Display: e = 0.06;c1 = [120 150 230]/255;c2 = ([120 150 230]+0)/383;c3 = ([120 150 230]+128)/383;patch([0 1 1 0],[0 0 1 1],c1);patch([0 1 1 1-e 1-e 0+e],[0 0 1 1-e 0+e 0+e],c2);patch([0 0 1 1-e 0+e 0+e],[0 1 1 1-e 1-e 0+e],c3);plot([0 1 1 0 0],[0 0 1 1 0]);disp('weights');
  "IW{2,1}(388,:)'" : Constant  Value=[-0.28470768213666742;-1.2796514465297362;-1.2221271411152648;0.25618557106785711;1.2967670557819968;0.36086682018748051;0.023047309676179843;0.42204305496930206;0.64625225792361962;0.27408710651131896]
      mask Display: e = 0.06;c1 = [120 150 230]/255;c2 = ([120 150 230]+0)/383;c3 = ([120 150 230]+128)/383;patch([0 1 1 0],[0 0 1 1],c1);patch([0 1 1 1-e 1-e 0+e],[0 0 1 1-e 0+e 0+e],c2);patch([0 0 1 1-e 0+e 0+e],[0 1 1 1-e 1-e 0+e],c3);plot([0 1 1 0 0],[0 0 1 1 0]);disp('weights');
  "IW{2,1}(389,:)'" : Constant  Value=[-0.089983281705121987;-0.84608344256757606;0.21849483330563546;0.24715733950872307;0.91264334235427991;0.40830919279730071;-0.39663238568113313;-0.17751544741641032;0.26737845571796803;-0.70630651090062269]
      mask Display: e = 0.06;c1 = [120 150 230]/255;c2 = ([120 150 230]+0)/383;c3 = ([120 150 230]+128)/383;patch([0 1 1 0],[0 0 1 1],c1);patch([0 1 1 1-e 1-e 0+e],[0 0 1 1-e 0+e 0+e],c2);patch([0 0 1 1-e 0+e 0+e],[0 1 1 1-e 1-e 0+e],c3);plot([0 1 1 0 0],[0 0 1 1 0]);disp('weights');
  "IW{2,1}(39,:)'" : Constant  Value=[0.83714116656432314;-0.28789832702947438;-1.0405415289472482;0.43838613871708854;0.6533170098909078;-0.22674123235297827;-0.70008559224105782;-0.215426487936179;-0.1141382181418133;0.54215887011952701]
      mask Display: e = 0.06;c1 = [120 150 230]/255;c2 = ([120 150 230]+0)/383;c3 = ([120 150 230]+128)/383;patch([0 1 1 0],[0 0 1 1],c1);patch([0 1 1 1-e 1-e 0+e],[0 0 1 1-e 0+e 0+e],c2);patch([0 0 1 1-e 0+e 0+e],[0 1 1 1-e 1-e 0+e],c3);plot([0 1 1 0 0],[0 0 1 1 0]);disp('weights');
  "IW{2,1}(390,:)'" : Constant  Value=[0.30793326590608083;-0.25605903974843758;0.66418825376186685;-0.2465588415760967;1.4972488753274904;0.13734840059190934;0.21668806597553103;0.43516296470234284;0.25348865712477542;0.19675010068052912]
      mask Display: e = 0.06;c1 = [120 150 230]/255;c2 = ([120 150 230]+0)/383;c3 = ([120 150 230]+128)/383;patch([0 1 1 0],[0 0 1 1],c1);patch([0 1 1 1-e 1-e 0+e],[0 0 1 1-e 0+e 0+e],c2);patch([0 0 1 1-e 0+e 0+e],[0 1 1 1-e 1-e 0+e],c3);plot([0 1 1 0 0],[0 0 1 1 0]);disp('weights');
  "IW{2,1}(391,:)'" : Constant  Value=[0.63344909186219922;0.26928420423960364;0.048665347165607997;0.28616878191427414;0.24772851739206869;0.089173857121743194;0.081454514690428526;0.082823257357263869;1.357003986477662;0.082616933473425358]
      mask Display: e = 0.06;c1 = [120 150 230]/255;c2 = ([120 150 230]+0)/383;c3 = ([120 150 230]+128)/383;patch([0 1 1 0],[0 0 1 1],c1);patch([0 1 1 1-e 1-e 0+e],[0 0 1 1-e 0+e 0+e],c2);patch([0 0 1 1-e 0+e 0+e],[0 1 1 1-e 1-e 0+e],c3);plot([0 1 1 0 0],[0 0 1 1 0]);disp('weights');
  "IW{2,1}(392,:)'" : Constant  Value=[-0.18179970817635177;-0.068562969878165084;-0.46188180773850757;-0.32585525549393318;-0.082580596353806046;0.3967450792615399;0.27660472848207912;1.0388917494596903;-0.50489454831165193;0.47026312179027219]
      mask Display: e = 0.06;c1 = [120 150 230]/255;c2 = ([120 150 230]+0)/383;c3 = ([120 150 230]+128)/383;patch([0 1 1 0],[0 0 1 1],c1);patch([0 1 1 1-e 1-e 0+e],[0 0 1 1-e 0+e 0+e],c2);patch([0 0 1 1-e 0+e 0+e],[0 1 1 1-e 1-e 0+e],c3);plot([0 1 1 0 0],[0 0 1 1 0]);disp('weights');
  "IW{2,1}(393,:)'" : Constant  Value=[0.69509326640789959;0.36564573378430776;0.37232212151915955;0.36344391440261747;-0.043888242673249311;0.34882089936244071;-0.55882332875909446;0.64002383406447294;-0.51206341444107295;0.43424718391911427]
      mask Display: e = 0.06;c1 = [120 150 230]/255;c2 = ([120 150 230]+0)/383;c3 = ([120 150 230]+128)/383;patch([0 1 1 0],[0 0 1 1],c1);patch([0 1 1 1-e 1-e 0+e],[0 0 1 1-e 0+e 0+e],c2);patch([0 0 1 1-e 0+e 0+e],[0 1 1 1-e 1-e 0+e],c3);plot([0 1 1 0 0],[0 0 1 1 0]);disp('weights');
  "IW{2,1}(394,:)'" : Constant  Value=[-0.54707569214968088;-1.1663687089192689;-0.70202859606470447;-0.46242643495916852;-0.14256967762415579;0.19569688115576178;0.042807372208786193;0.67307177336847746;-0.3213877301488704;0.0012939320972220614]
      mask Display: e = 0.06;c1 = [120 150 230]/255;c2 = ([120 150 230]+0)/383;c3 = ([120 150 230]+128)/383;patch([0 1 1 0],[0 0 1 1],c1);patch([0 1 1 1-e 1-e 0+e],[0 0 1 1-e 0+e 0+e],c2);patch([0 0 1 1-e 0+e 0+e],[0 1 1 1-e 1-e 0+e],c3);plot([0 1 1 0 0],[0 0 1 1 0]);disp('weights');
  "IW{2,1}(395,:)'" : Constant  Value=[0.12801122344869539;-0.67104375675680084;0.85473107975059404;-0.69992660567171927;0.35179898402244431;-0.21372571738989921;-1.0219155480323636;-0.35389775096443044;0.35514965175401492;-0.91353104197277679]
      mask Display: e = 0.06;c1 = [120 150 230]/255;c2 = ([120 150 230]+0)/383;c3 = ([120 150 230]+128)/383;patch([0 1 1 0],[0 0 1 1],c1);patch([0 1 1 1-e 1-e 0+e],[0 0 1 1-e 0+e 0+e],c2);patch([0 0 1 1-e 0+e 0+e],[0 1 1 1-e 1-e 0+e],c3);plot([0 1 1 0 0],[0 0 1 1 0]);disp('weights');
  "IW{2,1}(396,:)'" : Constant  Value=[0.28011993487630893;-0.032535386707143787;0.4992908801786089;-0.88612296753816233;-0.08997163855997764;0.012739655070945544;0.43044143325073392;-0.60354394171285275;1.3716299170443291;-1.1812421773946937]
      mask Display: e = 0.06;c1 = [120 150 230]/255;c2 = ([120 150 230]+0)/383;c3 = ([120 150 230]+128)/383;patch([0 1 1 0],[0 0 1 1],c1);patch([0 1 1 1-e 1-e 0+e],[0 0 1 1-e 0+e 0+e],c2);patch([0 0 1 1-e 0+e 0+e],[0 1 1 1-e 1-e 0+e],c3);plot([0 1 1 0 0],[0 0 1 1 0]);disp('weights');
  "IW{2,1}(397,:)'" : Constant  Value=[0.079598075852724215;-0.48549856546936276;0.72321593574995291;0.2513106444369857;1.246079257926175;0.44707186439544894;0.018105140364708783;0.24671460246309862;0.31292886481235721;-1.2093176271544437]
      mask Display: e = 0.06;c1 = [120 150 230]/255;c2 = ([120 150 230]+0)/383;c3 = ([120 150 230]+128)/383;patch([0 1 1 0],[0 0 1 1],c1);patch([0 1 1 1-e 1-e 0+e],[0 0 1 1-e 0+e 0+e],c2);patch([0 0 1 1-e 0+e 0+e],[0 1 1 1-e 1-e 0+e],c3);plot([0 1 1 0 0],[0 0 1 1 0]);disp('weights');
  "IW{2,1}(398,:)'" : Constant  Value=[-0.040523266254481008;-0.054967328439057037;-0.83206550636422105;-0.51073298166709735;0.53856329605258002;0.50047603638890448;-0.34476603678893536;0.23357285962735966;-0.084267247845521198;0.3274824535226199]
      mask Display: e = 0.06;c1 = [120 150 230]/255;c2 = ([120 150 230]+0)/383;c3 = ([120 150 230]+128)/383;patch([0 1 1 0],[0 0 1 1],c1);patch([0 1 1 1-e 1-e 0+e],[0 0 1 1-e 0+e 0+e],c2);patch([0 0 1 1-e 0+e 0+e],[0 1 1 1-e 1-e 0+e],c3);plot([0 1 1 0 0],[0 0 1 1 0]);disp('weights');
  "IW{2,1}(399,:)'" : Constant  Value=[-0.133394582106798;-0.7968871183789813;0.14069828992467939;0.1385020445243707;0.72971168474015335;0.75243682164172199;0.57085281531549503;0.18330839006805238;0.23581722568268468;0.16219392966106769]
      mask Display: e = 0.06;c1 = [120 150 230]/255;c2 = ([120 150 230]+0)/383;c3 = ([120 150 230]+128)/383;patch([0 1 1 0],[0 0 1 1],c1);patch([0 1 1 1-e 1-e 0+e],[0 0 1 1-e 0+e 0+e],c2);patch([0 0 1 1-e 0+e 0+e],[0 1 1 1-e 1-e 0+e],c3);plot([0 1 1 0 0],[0 0 1 1 0]);disp('weights');
  "IW{2,1}(4,:)'" : Constant  Value=[0.08296437556870298;-0.24180704508356449;-0.84505367905028672;0.24930925670189408;0.74672279566930477;0.58422529255872768;0.4627810852887646;-0.62375099396061662;0.56925388327469262;-0.77023153985394921]
      mask Display: e = 0.06;c1 = [120 150 230]/255;c2 = ([120 150 230]+0)/383;c3 = ([120 150 230]+128)/383;patch([0 1 1 0],[0 0 1 1],c1);patch([0 1 1 1-e 1-e 0+e],[0 0 1 1-e 0+e 0+e],c2);patch([0 0 1 1-e 0+e 0+e],[0 1 1 1-e 1-e 0+e],c3);plot([0 1 1 0 0],[0 0 1 1 0]);disp('weights');
  "IW{2,1}(40,:)'" : Constant  Value=[-0.17101324829756986;0.08216669814310823;-0.28095258190609956;-1.1001557176768548;0.42143570253746021;0.27018243611163861;0.41014869986522046;0.68432981210774502;0.031588140737934312;-0.091546956748061903]
      mask Display: e = 0.06;c1 = [120 150 230]/255;c2 = ([120 150 230]+0)/383;c3 = ([120 150 230]+128)/383;patch([0 1 1 0],[0 0 1 1],c1);patch([0 1 1 1-e 1-e 0+e],[0 0 1 1-e 0+e 0+e],c2);patch([0 0 1 1-e 0+e 0+e],[0 1 1 1-e 1-e 0+e],c3);plot([0 1 1 0 0],[0 0 1 1 0]);disp('weights');
  "IW{2,1}(400,:)'" : Constant  Value=[0.067579938778329171;-0.19135743134820038;-0.50123051187868328;0.11649406473084323;-0.45321423295075874;0.29577623461152197;-0.4977767316342035;0.24136926661870889;-0.4675562670591985;0.13943561939661647]
      mask Display: e = 0.06;c1 = [120 150 230]/255;c2 = ([120 150 230]+0)/383;c3 = ([120 150 230]+128)/383;patch([0 1 1 0],[0 0 1 1],c1);patch([0 1 1 1-e 1-e 0+e],[0 0 1 1-e 0+e 0+e],c2);patch([0 0 1 1-e 0+e 0+e],[0 1 1 1-e 1-e 0+e],c3);plot([0 1 1 0 0],[0 0 1 1 0]);disp('weights');
  "IW{2,1}(401,:)'" : Constant  Value=[-0.29522021854284353;-0.86848053786206203;-0.11816610878000566;-0.834103414105413;-0.66918118064807275;0.26962985734075506;0.4281344851755185;-0.015287272930904663;0.22277074180444972;-0.22488913167413865]
      mask Display: e = 0.06;c1 = [120 150 230]/255;c2 = ([120 150 230]+0)/383;c3 = ([120 150 230]+128)/383;patch([0 1 1 0],[0 0 1 1],c1);patch([0 1 1 1-e 1-e 0+e],[0 0 1 1-e 0+e 0+e],c2);patch([0 0 1 1-e 0+e 0+e],[0 1 1 1-e 1-e 0+e],c3);plot([0 1 1 0 0],[0 0 1 1 0]);disp('weights');
  "IW{2,1}(402,:)'" : Constant  Value=[0.6879758134544357;0.050774769481770878;1.1057766168553067;0.20975529310126947;-0.98877338926210545;0.62712882120042701;-0.45296832787695951;-0.47605557277901395;-0.068779973576777592;-0.54427873343798006]
      mask Display: e = 0.06;c1 = [120 150 230]/255;c2 = ([120 150 230]+0)/383;c3 = ([120 150 230]+128)/383;patch([0 1 1 0],[0 0 1 1],c1);patch([0 1 1 1-e 1-e 0+e],[0 0 1 1-e 0+e 0+e],c2);patch([0 0 1 1-e 0+e 0+e],[0 1 1 1-e 1-e 0+e],c3);plot([0 1 1 0 0],[0 0 1 1 0]);disp('weights');
  "IW{2,1}(403,:)'" : Constant  Value=[-0.11096791456958027;-1.1664367327553502;-0.75167536842129168;-0.15181692108110273;0.38718775459059468;0.22832632619413273;-0.047485606734524691;0.27852517545404376;-0.28512150382979384;-0.74712105311234689]
      mask Display: e = 0.06;c1 = [120 150 230]/255;c2 = ([120 150 230]+0)/383;c3 = ([120 150 230]+128)/383;patch([0 1 1 0],[0 0 1 1],c1);patch([0 1 1 1-e 1-e 0+e],[0 0 1 1-e 0+e 0+e],c2);patch([0 0 1 1-e 0+e 0+e],[0 1 1 1-e 1-e 0+e],c3);plot([0 1 1 0 0],[0 0 1 1 0]);disp('weights');
  "IW{2,1}(404,:)'" : Constant  Value=[0.77998916245455496;0.75269758786989738;-0.20300187523152596;-0.30735485354338205;0.55009959275356446;0.034300742227803327;-1.0922740138368829;-0.20343528530594018;-0.16367031369654766;-0.17849860737311984]
      mask Display: e = 0.06;c1 = [120 150 230]/255;c2 = ([120 150 230]+0)/383;c3 = ([120 150 230]+128)/383;patch([0 1 1 0],[0 0 1 1],c1);patch([0 1 1 1-e 1-e 0+e],[0 0 1 1-e 0+e 0+e],c2);patch([0 0 1 1-e 0+e 0+e],[0 1 1 1-e 1-e 0+e],c3);plot([0 1 1 0 0],[0 0 1 1 0]);disp('weights');
  "IW{2,1}(405,:)'" : Constant  Value=[0.73985140193634136;-0.40859180274287232;-0.66260311579689435;-0.15084085360292021;0.032487772986290242;-0.27962366117374804;-1.0637904944369065;0.2947374137268311;-0.45214843522537718;-1.2130272576345738]
      mask Display: e = 0.06;c1 = [120 150 230]/255;c2 = ([120 150 230]+0)/383;c3 = ([120 150 230]+128)/383;patch([0 1 1 0],[0 0 1 1],c1);patch([0 1 1 1-e 1-e 0+e],[0 0 1 1-e 0+e 0+e],c2);patch([0 0 1 1-e 0+e 0+e],[0 1 1 1-e 1-e 0+e],c3);plot([0 1 1 0 0],[0 0 1 1 0]);disp('weights');
  "IW{2,1}(41,:)'" : Constant  Value=[0.89937435097598506;0.0076924223842278205;0.04520516359203533;0.64404588882410507;0.24086477701989756;0.58800385045396109;0.41792909441939463;-0.23677621518619138;0.40010103701686905;-0.029654190352172233]
      mask Display: e = 0.06;c1 = [120 150 230]/255;c2 = ([120 150 230]+0)/383;c3 = ([120 150 230]+128)/383;patch([0 1 1 0],[0 0 1 1],c1);patch([0 1 1 1-e 1-e 0+e],[0 0 1 1-e 0+e 0+e],c2);patch([0 0 1 1-e 0+e 0+e],[0 1 1 1-e 1-e 0+e],c3);plot([0 1 1 0 0],[0 0 1 1 0]);disp('weights');
  "IW{2,1}(42,:)'" : Constant  Value=[-0.18304311782296523;-1.0287464009189853;-0.64772040348413984;0.24377249036643711;0.61652650701468192;0.48470484910273098;-0.050720117297440026;0.27385823152789751;-0.28646490361742827;-0.70037377342611784]
      mask Display: e = 0.06;c1 = [120 150 230]/255;c2 = ([120 150 230]+0)/383;c3 = ([120 150 230]+128)/383;patch([0 1 1 0],[0 0 1 1],c1);patch([0 1 1 1-e 1-e 0+e],[0 0 1 1-e 0+e 0+e],c2);patch([0 0 1 1-e 0+e 0+e],[0 1 1 1-e 1-e 0+e],c3);plot([0 1 1 0 0],[0 0 1 1 0]);disp('weights');
  "IW{2,1}(43,:)'" : Constant  Value=[-0.33275204604432601;-0.87682569386889797;0.52024703092329116;-0.91461872220735585;-0.17425654339616847;-0.35452086481617673;-1.2758942263979358;0.31684576431979389;-0.13582745386398254;-0.85005520178388694]
      mask Display: e = 0.06;c1 = [120 150 230]/255;c2 = ([120 150 230]+0)/383;c3 = ([120 150 230]+128)/383;patch([0 1 1 0],[0 0 1 1],c1);patch([0 1 1 1-e 1-e 0+e],[0 0 1 1-e 0+e 0+e],c2);patch([0 0 1 1-e 0+e 0+e],[0 1 1 1-e 1-e 0+e],c3);plot([0 1 1 0 0],[0 0 1 1 0]);disp('weights');
  "IW{2,1}(44,:)'" : Constant  Value=[-0.14663790510981192;-0.49462901299320905;0.68554699282010101;0.33408506872805549;-0.35203106375583049;0.59283363868442795;0.13890197885502648;-0.025368334809927118;0.97308034012406242;0.70947006749972275]
      mask Display: e = 0.06;c1 = [120 150 230]/255;c2 = ([120 150 230]+0)/383;c3 = ([120 150 230]+128)/383;patch([0 1 1 0],[0 0 1 1],c1);patch([0 1 1 1-e 1-e 0+e],[0 0 1 1-e 0+e 0+e],c2);patch([0 0 1 1-e 0+e 0+e],[0 1 1 1-e 1-e 0+e],c3);plot([0 1 1 0 0],[0 0 1 1 0]);disp('weights');
  "IW{2,1}(45,:)'" : Constant  Value=[0.89495055157338932;-0.78630498744429667;0.015195834684541637;0.31889360624268881;0.86256170812216215;-0.24489034803984688;-0.99278819569788646;0.59127529555623071;-0.51532164272744185;-0.32900237069725918]
      mask Display: e = 0.06;c1 = [120 150 230]/255;c2 = ([120 150 230]+0)/383;c3 = ([120 150 230]+128)/383;patch([0 1 1 0],[0 0 1 1],c1);patch([0 1 1 1-e 1-e 0+e],[0 0 1 1-e 0+e 0+e],c2);patch([0 0 1 1-e 0+e 0+e],[0 1 1 1-e 1-e 0+e],c3);plot([0 1 1 0 0],[0 0 1 1 0]);disp('weights');
  "IW{2,1}(46,:)'" : Constant  Value=[-0.094750878874135636;-0.63175876698559397;-0.39221309633492851;-0.066722832050202532;0.93297821828531891;0.41680878834233948;0.152872099587297;-0.15739052216154953;-0.28729072753486545;0.04684432073171757]
      mask Display: e = 0.06;c1 = [120 150 230]/255;c2 = ([120 150 230]+0)/383;c3 = ([120 150 230]+128)/383;patch([0 1 1 0],[0 0 1 1],c1);patch([0 1 1 1-e 1-e 0+e],[0 0 1 1-e 0+e 0+e],c2);patch([0 0 1 1-e 0+e 0+e],[0 1 1 1-e 1-e 0+e],c3);plot([0 1 1 0 0],[0 0 1 1 0]);disp('weights');
  "IW{2,1}(47,:)'" : Constant  Value=[1.5956697795708239;-0.4771235476782909;-0.12195547091325162;0.13103316964172379;-0.34888925402337961;-0.41288175937927774;-0.074861921347058533;0.4836041854180001;0.75858201938977765;-0.80707188813929132]
      mask Display: e = 0.06;c1 = [120 150 230]/255;c2 = ([120 150 230]+0)/383;c3 = ([120 150 230]+128)/383;patch([0 1 1 0],[0 0 1 1],c1);patch([0 1 1 1-e 1-e 0+e],[0 0 1 1-e 0+e 0+e],c2);patch([0 0 1 1-e 0+e 0+e],[0 1 1 1-e 1-e 0+e],c3);plot([0 1 1 0 0],[0 0 1 1 0]);disp('weights');
  "IW{2,1}(48,:)'" : Constant  Value=[0.28404975677496269;-0.178995256584534;-0.96602088085074844;-0.19923617656618439;-0.040269901918144335;-0.060546675638951719;-0.029270092207745679;0.11899785338880206;0.32570357212099071;0.50971482853963468]
      mask Display: e = 0.06;c1 = [120 150 230]/255;c2 = ([120 150 230]+0)/383;c3 = ([120 150 230]+128)/383;patch([0 1 1 0],[0 0 1 1],c1);patch([0 1 1 1-e 1-e 0+e],[0 0 1 1-e 0+e 0+e],c2);patch([0 0 1 1-e 0+e 0+e],[0 1 1 1-e 1-e 0+e],c3);plot([0 1 1 0 0],[0 0 1 1 0]);disp('weights');
  "IW{2,1}(49,:)'" : Constant  Value=[0.11025656435855408;-0.19726013771415735;-0.80163671290734162;-0.63260382364143053;-0.94122577418786091;0.23480559280453572;-0.049347464515737835;-0.5433593259044146;0.71353794782121682;-0.20031911832940991]
      mask Display: e = 0.06;c1 = [120 150 230]/255;c2 = ([120 150 230]+0)/383;c3 = ([120 150 230]+128)/383;patch([0 1 1 0],[0 0 1 1],c1);patch([0 1 1 1-e 1-e 0+e],[0 0 1 1-e 0+e 0+e],c2);patch([0 0 1 1-e 0+e 0+e],[0 1 1 1-e 1-e 0+e],c3);plot([0 1 1 0 0],[0 0 1 1 0]);disp('weights');
  "IW{2,1}(5,:)'" : Constant  Value=[-0.52500191515971684;-0.181365053603458;0.27184213961323417;-0.69821436581091767;-0.47667921947017666;0.41828542464578011;-0.37839212885083895;-0.013431798998805353;0.34436648600710634;0.08819800384300587]
      mask Display: e = 0.06;c1 = [120 150 230]/255;c2 = ([120 150 230]+0)/383;c3 = ([120 150 230]+128)/383;patch([0 1 1 0],[0 0 1 1],c1);patch([0 1 1 1-e 1-e 0+e],[0 0 1 1-e 0+e 0+e],c2);patch([0 0 1 1-e 0+e 0+e],[0 1 1 1-e 1-e 0+e],c3);plot([0 1 1 0 0],[0 0 1 1 0]);disp('weights');
  "IW{2,1}(50,:)'" : Constant  Value=[0.69107290696923507;0.072377655786278083;-0.98288051217865358;-0.37604251737202438;1.0267399312353049;0.17164583570332145;-0.63776120138720882;0.013150538292690084;-0.11968483657434481;0.86312033057009341]
      mask Display: e = 0.06;c1 = [120 150 230]/255;c2 = ([120 150 230]+0)/383;c3 = ([120 150 230]+128)/383;patch([0 1 1 0],[0 0 1 1],c1);patch([0 1 1 1-e 1-e 0+e],[0 0 1 1-e 0+e 0+e],c2);patch([0 0 1 1-e 0+e 0+e],[0 1 1 1-e 1-e 0+e],c3);plot([0 1 1 0 0],[0 0 1 1 0]);disp('weights');
  "IW{2,1}(51,:)'" : Constant  Value=[-0.22044007034332685;-0.92332773281010083;0.41919473528232387;0.023900699612631748;0.63243141570214279;0.80662317898666425;0.17985892401295142;0.49912432578251564;-0.30221848555253572;-0.61493078452366423]
      mask Display: e = 0.06;c1 = [120 150 230]/255;c2 = ([120 150 230]+0)/383;c3 = ([120 150 230]+128)/383;patch([0 1 1 0],[0 0 1 1],c1);patch([0 1 1 1-e 1-e 0+e],[0 0 1 1-e 0+e 0+e],c2);patch([0 0 1 1-e 0+e 0+e],[0 1 1 1-e 1-e 0+e],c3);plot([0 1 1 0 0],[0 0 1 1 0]);disp('weights');
  "IW{2,1}(52,:)'" : Constant  Value=[0.45833871077634464;0.34464150537555299;0.11157589334294676;-0.75403678542852726;0.85414186794864222;0.25111988098708249;-0.19668692002006607;0.53733453162067946;0.058181674637455605;-0.0044757717304228506]
      mask Display: e = 0.06;c1 = [120 150 230]/255;c2 = ([120 150 230]+0)/383;c3 = ([120 150 230]+128)/383;patch([0 1 1 0],[0 0 1 1],c1);patch([0 1 1 1-e 1-e 0+e],[0 0 1 1-e 0+e 0+e],c2);patch([0 0 1 1-e 0+e 0+e],[0 1 1 1-e 1-e 0+e],c3);plot([0 1 1 0 0],[0 0 1 1 0]);disp('weights');
  "IW{2,1}(53,:)'" : Constant  Value=[0.7636460777580143;-0.61299356189326248;-0.12571281474699489;0.68989078251054148;0.67189089007792335;0.19463720924934078;-0.77077099968741691;0.2004747502754399;-0.94956582166829373;0.36301569007059165]
      mask Display: e = 0.06;c1 = [120 150 230]/255;c2 = ([120 150 230]+0)/383;c3 = ([120 150 230]+128)/383;patch([0 1 1 0],[0 0 1 1],c1);patch([0 1 1 1-e 1-e 0+e],[0 0 1 1-e 0+e 0+e],c2);patch([0 0 1 1-e 0+e 0+e],[0 1 1 1-e 1-e 0+e],c3);plot([0 1 1 0 0],[0 0 1 1 0]);disp('weights');
  "IW{2,1}(54,:)'" : Constant  Value=[0.62781243882554938;-0.5065266699076314;0.24896970760203069;0.5343092920057716;0.60829027030319682;0.090008219320647176;0.10145308640950917;0.36407851230102711;0.61890402128583233;-0.044900810840943328]
      mask Display: e = 0.06;c1 = [120 150 230]/255;c2 = ([120 150 230]+0)/383;c3 = ([120 150 230]+128)/383;patch([0 1 1 0],[0 0 1 1],c1);patch([0 1 1 1-e 1-e 0+e],[0 0 1 1-e 0+e 0+e],c2);patch([0 0 1 1-e 0+e 0+e],[0 1 1 1-e 1-e 0+e],c3);plot([0 1 1 0 0],[0 0 1 1 0]);disp('weights');
  "IW{2,1}(55,:)'" : Constant  Value=[0.45066932251101871;-0.82497263443814339;0.2585168828378126;0.36846081422245253;-0.017414293841225587;0.1414967216231594;-0.2662662924514283;0.29129960448753101;0.36716802017241085;-0.40032117942323076]
      mask Display: e = 0.06;c1 = [120 150 230]/255;c2 = ([120 150 230]+0)/383;c3 = ([120 150 230]+128)/383;patch([0 1 1 0],[0 0 1 1],c1);patch([0 1 1 1-e 1-e 0+e],[0 0 1 1-e 0+e 0+e],c2);patch([0 0 1 1-e 0+e 0+e],[0 1 1 1-e 1-e 0+e],c3);plot([0 1 1 0 0],[0 0 1 1 0]);disp('weights');
  "IW{2,1}(56,:)'" : Constant  Value=[-0.71244090374714031;0.14928060642448823;0.74304668868590562;-0.95778185667768145;-0.51553109074282133;1.0439163624132795;0.50765493894189395;0.5263873823695292;0.59998450088238631;-1.0832594721802185]
      mask Display: e = 0.06;c1 = [120 150 230]/255;c2 = ([120 150 230]+0)/383;c3 = ([120 150 230]+128)/383;patch([0 1 1 0],[0 0 1 1],c1);patch([0 1 1 1-e 1-e 0+e],[0 0 1 1-e 0+e 0+e],c2);patch([0 0 1 1-e 0+e 0+e],[0 1 1 1-e 1-e 0+e],c3);plot([0 1 1 0 0],[0 0 1 1 0]);disp('weights');
  "IW{2,1}(57,:)'" : Constant  Value=[-0.16538674937293768;-1.1888774879353763;0.032097917706363138;0.55628007185118333;1.1426909323529186;0.32659488207074516;0.47485841116846539;-0.27020548545565909;0.88198733168081933;-0.74765002684160486]
      mask Display: e = 0.06;c1 = [120 150 230]/255;c2 = ([120 150 230]+0)/383;c3 = ([120 150 230]+128)/383;patch([0 1 1 0],[0 0 1 1],c1);patch([0 1 1 1-e 1-e 0+e],[0 0 1 1-e 0+e 0+e],c2);patch([0 0 1 1-e 0+e 0+e],[0 1 1 1-e 1-e 0+e],c3);plot([0 1 1 0 0],[0 0 1 1 0]);disp('weights');
  "IW{2,1}(58,:)'" : Constant  Value=[-0.023773644854532955;0.59932756323559599;-0.19970415139329928;-0.62777108222091138;0.94924190713151002;0.88186525040478703;-0.39835452524768894;-0.03025826028316797;-0.5269323269402294;0.77021216222237632]
      mask Display: e = 0.06;c1 = [120 150 230]/255;c2 = ([120 150 230]+0)/383;c3 = ([120 150 230]+128)/383;patch([0 1 1 0],[0 0 1 1],c1);patch([0 1 1 1-e 1-e 0+e],[0 0 1 1-e 0+e 0+e],c2);patch([0 0 1 1-e 0+e 0+e],[0 1 1 1-e 1-e 0+e],c3);plot([0 1 1 0 0],[0 0 1 1 0]);disp('weights');
  "IW{2,1}(59,:)'" : Constant  Value=[-0.54415225662389699;-0.80245767289365244;0.24231426418852037;0.38482423703237856;0.67500766538217483;0.48783296194514969;-0.66657997050107431;-0.10526936322941566;-0.70456411053205747;0.39025582005048776]
      mask Display: e = 0.06;c1 = [120 150 230]/255;c2 = ([120 150 230]+0)/383;c3 = ([120 150 230]+128)/383;patch([0 1 1 0],[0 0 1 1],c1);patch([0 1 1 1-e 1-e 0+e],[0 0 1 1-e 0+e 0+e],c2);patch([0 0 1 1-e 0+e 0+e],[0 1 1 1-e 1-e 0+e],c3);plot([0 1 1 0 0],[0 0 1 1 0]);disp('weights');
  "IW{2,1}(6,:)'" : Constant  Value=[-0.42782719672099162;-0.53921723226502438;0.42738356994875798;-0.29653061129783459;-1.1299448948898834;0.39945129472724672;-0.64944087381054927;-0.43183258294883647;0.075909567771779665;-0.26470116370216223]
      mask Display: e = 0.06;c1 = [120 150 230]/255;c2 = ([120 150 230]+0)/383;c3 = ([120 150 230]+128)/383;patch([0 1 1 0],[0 0 1 1],c1);patch([0 1 1 1-e 1-e 0+e],[0 0 1 1-e 0+e 0+e],c2);patch([0 0 1 1-e 0+e 0+e],[0 1 1 1-e 1-e 0+e],c3);plot([0 1 1 0 0],[0 0 1 1 0]);disp('weights');
  "IW{2,1}(60,:)'" : Constant  Value=[0.10998049653071873;-0.96269425400316833;0.3157894070243758;-0.38104602068458748;-0.05505195477299768;-0.52422190058137852;-0.99867558318877092;-0.12352918099037863;-0.011359751115228689;-0.29117030710622915]
      mask Display: e = 0.06;c1 = [120 150 230]/255;c2 = ([120 150 230]+0)/383;c3 = ([120 150 230]+128)/383;patch([0 1 1 0],[0 0 1 1],c1);patch([0 1 1 1-e 1-e 0+e],[0 0 1 1-e 0+e 0+e],c2);patch([0 0 1 1-e 0+e 0+e],[0 1 1 1-e 1-e 0+e],c3);plot([0 1 1 0 0],[0 0 1 1 0]);disp('weights');
  "IW{2,1}(61,:)'" : Constant  Value=[-0.35121660594401088;-0.4792442817940496;0.6158680096375837;-0.33994951516579447;0.33342723080950265;0.40154623053864841;0.3974361193261321;0.45531290909009725;0.99518636084403367;0.34758170214403628]
      mask Display: e = 0.06;c1 = [120 150 230]/255;c2 = ([120 150 230]+0)/383;c3 = ([120 150 230]+128)/383;patch([0 1 1 0],[0 0 1 1],c1);patch([0 1 1 1-e 1-e 0+e],[0 0 1 1-e 0+e 0+e],c2);patch([0 0 1 1-e 0+e 0+e],[0 1 1 1-e 1-e 0+e],c3);plot([0 1 1 0 0],[0 0 1 1 0]);disp('weights');
  "IW{2,1}(62,:)'" : Constant  Value=[-0.79526448424360707;-0.58655833806673552;0.80790665960649544;-0.51274468967053211;0.58751412833993311;0.74517964504534218;0.39032786772911898;0.25200603036470653;0.6369425321080604;0.00095791149327584257]
      mask Display: e = 0.06;c1 = [120 150 230]/255;c2 = ([120 150 230]+0)/383;c3 = ([120 150 230]+128)/383;patch([0 1 1 0],[0 0 1 1],c1);patch([0 1 1 1-e 1-e 0+e],[0 0 1 1-e 0+e 0+e],c2);patch([0 0 1 1-e 0+e 0+e],[0 1 1 1-e 1-e 0+e],c3);plot([0 1 1 0 0],[0 0 1 1 0]);disp('weights');
  "IW{2,1}(63,:)'" : Constant  Value=[-0.17944547588828524;-1.156513382530963;-0.21115377320473763;-0.27798713333957664;-0.30362916802035683;0.0089912759893863159;-0.20161856099174005;-0.29340784044670437;0.12091124464431183;-0.84958151880670341]
      mask Display: e = 0.06;c1 = [120 150 230]/255;c2 = ([120 150 230]+0)/383;c3 = ([120 150 230]+128)/383;patch([0 1 1 0],[0 0 1 1],c1);patch([0 1 1 1-e 1-e 0+e],[0 0 1 1-e 0+e 0+e],c2);patch([0 0 1 1-e 0+e 0+e],[0 1 1 1-e 1-e 0+e],c3);plot([0 1 1 0 0],[0 0 1 1 0]);disp('weights');
  "IW{2,1}(64,:)'" : Constant  Value=[0.57355571900112867;-0.8322528426332656;0.27641707876591265;0.30118331809855897;-0.39863824319699509;-0.23993380091376926;-0.57397260900270486;0.52131353388493928;-0.20292978143515825;-0.23626097806361279]
      mask Display: e = 0.06;c1 = [120 150 230]/255;c2 = ([120 150 230]+0)/383;c3 = ([120 150 230]+128)/383;patch([0 1 1 0],[0 0 1 1],c1);patch([0 1 1 1-e 1-e 0+e],[0 0 1 1-e 0+e 0+e],c2);patch([0 0 1 1-e 0+e 0+e],[0 1 1 1-e 1-e 0+e],c3);plot([0 1 1 0 0],[0 0 1 1 0]);disp('weights');
  "IW{2,1}(65,:)'" : Constant  Value=[0.47044309546476726;0.35648970674839797;0.22457831389431818;-1.2017818535539146;-0.20684242225378976;0.36811403264928994;0.060183735665818;0.50159833261081932;-0.36168050036341842;-0.83349026594917386]
      mask Display: e = 0.06;c1 = [120 150 230]/255;c2 = ([120 150 230]+0)/383;c3 = ([120 150 230]+128)/383;patch([0 1 1 0],[0 0 1 1],c1);patch([0 1 1 1-e 1-e 0+e],[0 0 1 1-e 0+e 0+e],c2);patch([0 0 1 1-e 0+e 0+e],[0 1 1 1-e 1-e 0+e],c3);plot([0 1 1 0 0],[0 0 1 1 0]);disp('weights');
  "IW{2,1}(66,:)'" : Constant  Value=[-0.091440476718846142;-0.18611976021165264;0.37917495803373247;-0.3619246008211483;-0.28134206850186305;0.77213934079861579;0.044392369405719737;0.53280179084557777;-0.76412687976319726;0.83921279939789717]
      mask Display: e = 0.06;c1 = [120 150 230]/255;c2 = ([120 150 230]+0)/383;c3 = ([120 150 230]+128)/383;patch([0 1 1 0],[0 0 1 1],c1);patch([0 1 1 1-e 1-e 0+e],[0 0 1 1-e 0+e 0+e],c2);patch([0 0 1 1-e 0+e 0+e],[0 1 1 1-e 1-e 0+e],c3);plot([0 1 1 0 0],[0 0 1 1 0]);disp('weights');
  "IW{2,1}(67,:)'" : Constant  Value=[0.43016724727989553;-0.29361093508867764;-0.33745368531818037;0.094489461305739597;-0.68281360268910207;0.7074691309568103;0.39059159938954313;0.74007393144217182;-0.098063724245145617;1.2998638714551476]
      mask Display: e = 0.06;c1 = [120 150 230]/255;c2 = ([120 150 230]+0)/383;c3 = ([120 150 230]+128)/383;patch([0 1 1 0],[0 0 1 1],c1);patch([0 1 1 1-e 1-e 0+e],[0 0 1 1-e 0+e 0+e],c2);patch([0 0 1 1-e 0+e 0+e],[0 1 1 1-e 1-e 0+e],c3);plot([0 1 1 0 0],[0 0 1 1 0]);disp('weights');
  "IW{2,1}(68,:)'" : Constant  Value=[0.35585835905521901;0.42627712377518057;0.13301214646746129;0.34173440176350239;-0.47111552806424473;0.85735458487343208;0.32110880382104806;-0.14878343079915662;-0.017104624387671463;0.22064395893928113]
      mask Display: e = 0.06;c1 = [120 150 230]/255;c2 = ([120 150 230]+0)/383;c3 = ([120 150 230]+128)/383;patch([0 1 1 0],[0 0 1 1],c1);patch([0 1 1 1-e 1-e 0+e],[0 0 1 1-e 0+e 0+e],c2);patch([0 0 1 1-e 0+e 0+e],[0 1 1 1-e 1-e 0+e],c3);plot([0 1 1 0 0],[0 0 1 1 0]);disp('weights');
  "IW{2,1}(69,:)'" : Constant  Value=[0.33318925046250281;-0.31988885692149432;-1.1847586623559354;0.057036474936227773;0.17611122029075429;0.50792618284244029;-0.22904493841638146;0.34288614544499646;-0.66950330141204573;0.57321443780994408]
      mask Display: e = 0.06;c1 = [120 150 230]/255;c2 = ([120 150 230]+0)/383;c3 = ([120 150 230]+128)/383;patch([0 1 1 0],[0 0 1 1],c1);patch([0 1 1 1-e 1-e 0+e],[0 0 1 1-e 0+e 0+e],c2);patch([0 0 1 1-e 0+e 0+e],[0 1 1 1-e 1-e 0+e],c3);plot([0 1 1 0 0],[0 0 1 1 0]);disp('weights');
  "IW{2,1}(7,:)'" : Constant  Value=[0.50157802911375649;0.37764160145304082;0.055377822051641545;-0.015577512997780818;0.37707173753925521;0.65656264193933578;0.18996388289176341;0.42952686209355384;-0.29449426929162015;0.87071809211777063]
      mask Display: e = 0.06;c1 = [120 150 230]/255;c2 = ([120 150 230]+0)/383;c3 = ([120 150 230]+128)/383;patch([0 1 1 0],[0 0 1 1],c1);patch([0 1 1 1-e 1-e 0+e],[0 0 1 1-e 0+e 0+e],c2);patch([0 0 1 1-e 0+e 0+e],[0 1 1 1-e 1-e 0+e],c3);plot([0 1 1 0 0],[0 0 1 1 0]);disp('weights');
  "IW{2,1}(70,:)'" : Constant  Value=[0.48380306451682126;-0.26730364402643564;-0.51413390118584446;-0.15593003025452573;-0.81920536236780361;0.24507122479122601;-0.073201240193239897;0.39513648695408732;-0.49731176598443344;0.32269463023598577]
      mask Display: e = 0.06;c1 = [120 150 230]/255;c2 = ([120 150 230]+0)/383;c3 = ([120 150 230]+128)/383;patch([0 1 1 0],[0 0 1 1],c1);patch([0 1 1 1-e 1-e 0+e],[0 0 1 1-e 0+e 0+e],c2);patch([0 0 1 1-e 0+e 0+e],[0 1 1 1-e 1-e 0+e],c3);plot([0 1 1 0 0],[0 0 1 1 0]);disp('weights');
  "IW{2,1}(71,:)'" : Constant  Value=[0.73715437642379833;-0.25974655814015735;0.72688158634557898;0.88438231853130467;-0.048457821861365658;0.62537408458899058;-0.73475005253693104;0.36871116716615865;-0.20814381487234024;-0.39680728514968661]
      mask Display: e = 0.06;c1 = [120 150 230]/255;c2 = ([120 150 230]+0)/383;c3 = ([120 150 230]+128)/383;patch([0 1 1 0],[0 0 1 1],c1);patch([0 1 1 1-e 1-e 0+e],[0 0 1 1-e 0+e 0+e],c2);patch([0 0 1 1-e 0+e 0+e],[0 1 1 1-e 1-e 0+e],c3);plot([0 1 1 0 0],[0 0 1 1 0]);disp('weights');
  "IW{2,1}(72,:)'" : Constant  Value=[0.69473012529740075;0.6755124789922391;0.21654571383821083;0.33324316856314473;0.64568639013368645;0.78487041650421729;-0.487708527043486;-0.17701559033191636;0.42402716320381112;0.26143167065287054]
      mask Display: e = 0.06;c1 = [120 150 230]/255;c2 = ([120 150 230]+0)/383;c3 = ([120 150 230]+128)/383;patch([0 1 1 0],[0 0 1 1],c1);patch([0 1 1 1-e 1-e 0+e],[0 0 1 1-e 0+e 0+e],c2);patch([0 0 1 1-e 0+e 0+e],[0 1 1 1-e 1-e 0+e],c3);plot([0 1 1 0 0],[0 0 1 1 0]);disp('weights');
  "IW{2,1}(73,:)'" : Constant  Value=[0.59719756210752584;-0.39990067840313803;0.060174677993690834;1.0721176791174669;1.0011067065664874;0.75764024484071268;0.44172954832253464;0.080295434290404533;0.078531885463810264;0.24239051478149917]
      mask Display: e = 0.06;c1 = [120 150 230]/255;c2 = ([120 150 230]+0)/383;c3 = ([120 150 230]+128)/383;patch([0 1 1 0],[0 0 1 1],c1);patch([0 1 1 1-e 1-e 0+e],[0 0 1 1-e 0+e 0+e],c2);patch([0 0 1 1-e 0+e 0+e],[0 1 1 1-e 1-e 0+e],c3);plot([0 1 1 0 0],[0 0 1 1 0]);disp('weights');
  "IW{2,1}(74,:)'" : Constant  Value=[-0.081047125321045133;-0.63924884030106999;-0.60360658407151491;-0.67612930836824958;0.39577609310357675;-0.28690217042006372;-0.87279928311190291;-0.48836718950542124;-0.14317722093925445;-0.12145095675108741]
      mask Display: e = 0.06;c1 = [120 150 230]/255;c2 = ([120 150 230]+0)/383;c3 = ([120 150 230]+128)/383;patch([0 1 1 0],[0 0 1 1],c1);patch([0 1 1 1-e 1-e 0+e],[0 0 1 1-e 0+e 0+e],c2);patch([0 0 1 1-e 0+e 0+e],[0 1 1 1-e 1-e 0+e],c3);plot([0 1 1 0 0],[0 0 1 1 0]);disp('weights');
  "IW{2,1}(75,:)'" : Constant  Value=[0.88806631547243453;-0.64917709648831678;-0.45250922069781108;0.10422752718025158;0.19398261311597961;-0.43310899909095324;-1.1570748607538723;-0.072652136071218149;-0.34134703372482533;-0.17829569043500598]
      mask Display: e = 0.06;c1 = [120 150 230]/255;c2 = ([120 150 230]+0)/383;c3 = ([120 150 230]+128)/383;patch([0 1 1 0],[0 0 1 1],c1);patch([0 1 1 1-e 1-e 0+e],[0 0 1 1-e 0+e 0+e],c2);patch([0 0 1 1-e 0+e 0+e],[0 1 1 1-e 1-e 0+e],c3);plot([0 1 1 0 0],[0 0 1 1 0]);disp('weights');
  "IW{2,1}(76,:)'" : Constant  Value=[0.83524180398494896;-0.49092034624206876;-0.38960669291361927;0.232563657802074;0.78065574919800107;0.29748284058073821;0.40208833353056372;-0.64065831559731334;1.0449573168563655;-0.49140079517398516]
      mask Display: e = 0.06;c1 = [120 150 230]/255;c2 = ([120 150 230]+0)/383;c3 = ([120 150 230]+128)/383;patch([0 1 1 0],[0 0 1 1],c1);patch([0 1 1 1-e 1-e 0+e],[0 0 1 1-e 0+e 0+e],c2);patch([0 0 1 1-e 0+e 0+e],[0 1 1 1-e 1-e 0+e],c3);plot([0 1 1 0 0],[0 0 1 1 0]);disp('weights');
  "IW{2,1}(77,:)'" : Constant  Value=[0.30417007746436076;0.26591885150952932;0.71978931452130313;-0.40172829738116833;0.12559439352547419;-0.045965978884079495;-0.4133109012211264;0.013999861135959912;0.48259055184592298;-0.43139152447364226]
      mask Display: e = 0.06;c1 = [120 150 230]/255;c2 = ([120 150 230]+0)/383;c3 = ([120 150 230]+128)/383;patch([0 1 1 0],[0 0 1 1],c1);patch([0 1 1 1-e 1-e 0+e],[0 0 1 1-e 0+e 0+e],c2);patch([0 0 1 1-e 0+e 0+e],[0 1 1 1-e 1-e 0+e],c3);plot([0 1 1 0 0],[0 0 1 1 0]);disp('weights');
  "IW{2,1}(78,:)'" : Constant  Value=[0.12921031222725632;0.17183587934950229;0.71649367291425858;-0.61949173379836231;0.004184726911171055;0.26680588035967556;-0.22119240716476085;-0.057994173830689416;-0.077552202900456613;-0.76956618456766068]
      mask Display: e = 0.06;c1 = [120 150 230]/255;c2 = ([120 150 230]+0)/383;c3 = ([120 150 230]+128)/383;patch([0 1 1 0],[0 0 1 1],c1);patch([0 1 1 1-e 1-e 0+e],[0 0 1 1-e 0+e 0+e],c2);patch([0 0 1 1-e 0+e 0+e],[0 1 1 1-e 1-e 0+e],c3);plot([0 1 1 0 0],[0 0 1 1 0]);disp('weights');
  "IW{2,1}(79,:)'" : Constant  Value=[-0.11480897084710617;-1.2738342086137671;-0.22231141577199975;0.23652628228792391;-0.36263667881107009;0.10521516278662263;0.59894306174693457;0.73051866293776557;0.98334552218294458;0.28169875368619129]
      mask Display: e = 0.06;c1 = [120 150 230]/255;c2 = ([120 150 230]+0)/383;c3 = ([120 150 230]+128)/383;patch([0 1 1 0],[0 0 1 1],c1);patch([0 1 1 1-e 1-e 0+e],[0 0 1 1-e 0+e 0+e],c2);patch([0 0 1 1-e 0+e 0+e],[0 1 1 1-e 1-e 0+e],c3);plot([0 1 1 0 0],[0 0 1 1 0]);disp('weights');
  "IW{2,1}(8,:)'" : Constant  Value=[0.3403961876196494;-0.48546724556322746;-0.81297062755575833;0.22767303895908514;0.21330536018951057;0.025602410164580279;-0.34066784319951138;-0.42011494445623493;0.70706888946338298;0.77671567063730684]
      mask Display: e = 0.06;c1 = [120 150 230]/255;c2 = ([120 150 230]+0)/383;c3 = ([120 150 230]+128)/383;patch([0 1 1 0],[0 0 1 1],c1);patch([0 1 1 1-e 1-e 0+e],[0 0 1 1-e 0+e 0+e],c2);patch([0 0 1 1-e 0+e 0+e],[0 1 1 1-e 1-e 0+e],c3);plot([0 1 1 0 0],[0 0 1 1 0]);disp('weights');
  "IW{2,1}(80,:)'" : Constant  Value=[0.37528035854945258;-0.31178305997729716;0.63265598940820977;0.56910005220993287;0.61160074268188358;0.18067758462514699;-0.71583620760820565;-0.59826190377065369;0.7097392303916763;0.13859365829274908]
      mask Display: e = 0.06;c1 = [120 150 230]/255;c2 = ([120 150 230]+0)/383;c3 = ([120 150 230]+128)/383;patch([0 1 1 0],[0 0 1 1],c1);patch([0 1 1 1-e 1-e 0+e],[0 0 1 1-e 0+e 0+e],c2);patch([0 0 1 1-e 0+e 0+e],[0 1 1 1-e 1-e 0+e],c3);plot([0 1 1 0 0],[0 0 1 1 0]);disp('weights');
  "IW{2,1}(81,:)'" : Constant  Value=[-0.58793073454306821;-0.26816393947911532;0.56190702676396875;-0.47506493968695196;-0.89854985340265381;0.85293265031530385;0.2903301251508501;0.22699241518584501;0.53356147768829321;0.52739654056512542]
      mask Display: e = 0.06;c1 = [120 150 230]/255;c2 = ([120 150 230]+0)/383;c3 = ([120 150 230]+128)/383;patch([0 1 1 0],[0 0 1 1],c1);patch([0 1 1 1-e 1-e 0+e],[0 0 1 1-e 0+e 0+e],c2);patch([0 0 1 1-e 0+e 0+e],[0 1 1 1-e 1-e 0+e],c3);plot([0 1 1 0 0],[0 0 1 1 0]);disp('weights');
  "IW{2,1}(82,:)'" : Constant  Value=[0.88249934078984738;0.95639002854877475;-0.11002428199681158;-0.17395484366496358;-0.49778544530843644;0.58996533226190029;-0.18046738207809715;-0.13387435050662494;-0.044683105569553627;0.52707937754223722]
      mask Display: e = 0.06;c1 = [120 150 230]/255;c2 = ([120 150 230]+0)/383;c3 = ([120 150 230]+128)/383;patch([0 1 1 0],[0 0 1 1],c1);patch([0 1 1 1-e 1-e 0+e],[0 0 1 1-e 0+e 0+e],c2);patch([0 0 1 1-e 0+e 0+e],[0 1 1 1-e 1-e 0+e],c3);plot([0 1 1 0 0],[0 0 1 1 0]);disp('weights');
  "IW{2,1}(83,:)'" : Constant  Value=[0.17401538546537959;0.14959031299170569;-1.0169316754468576;0.37982343637671845;1.1164666529921523;0.88585101835562174;0.15533537141992243;-0.29505417638278397;0.037254566282094226;-0.005548589917322877]
      mask Display: e = 0.06;c1 = [120 150 230]/255;c2 = ([120 150 230]+0)/383;c3 = ([120 150 230]+128)/383;patch([0 1 1 0],[0 0 1 1],c1);patch([0 1 1 1-e 1-e 0+e],[0 0 1 1-e 0+e 0+e],c2);patch([0 0 1 1-e 0+e 0+e],[0 1 1 1-e 1-e 0+e],c3);plot([0 1 1 0 0],[0 0 1 1 0]);disp('weights');
  "IW{2,1}(84,:)'" : Constant  Value=[1.100497701625363;-0.28113962046103347;-0.74072234756280297;0.86713467243732034;1.2413050122198648;0.0080247191640926419;-0.48728829873168145;-0.7964953486481321;0.94364522828210484;0.49113603313291504]
      mask Display: e = 0.06;c1 = [120 150 230]/255;c2 = ([120 150 230]+0)/383;c3 = ([120 150 230]+128)/383;patch([0 1 1 0],[0 0 1 1],c1);patch([0 1 1 1-e 1-e 0+e],[0 0 1 1-e 0+e 0+e],c2);patch([0 0 1 1-e 0+e 0+e],[0 1 1 1-e 1-e 0+e],c3);plot([0 1 1 0 0],[0 0 1 1 0]);disp('weights');
  "IW{2,1}(85,:)'" : Constant  Value=[0.80215788233574137;-0.058770655656507853;0.30624990171668842;0.57726726375296167;1.5591060716994432;0.052643665430780917;0.017738325164090074;0.88100372072728195;-0.21732429361670613;-0.72236655378901538]
      mask Display: e = 0.06;c1 = [120 150 230]/255;c2 = ([120 150 230]+0)/383;c3 = ([120 150 230]+128)/383;patch([0 1 1 0],[0 0 1 1],c1);patch([0 1 1 1-e 1-e 0+e],[0 0 1 1-e 0+e 0+e],c2);patch([0 0 1 1-e 0+e 0+e],[0 1 1 1-e 1-e 0+e],c3);plot([0 1 1 0 0],[0 0 1 1 0]);disp('weights');
  "IW{2,1}(86,:)'" : Constant  Value=[0.618882737160945;0.23121463630736142;-0.24153582482761282;-0.24633794156939137;-0.89894441841684514;0.41867762224084126;-0.16587608226150116;-0.50894007958410237;0.74892215462681211;-0.096336266747773014]
      mask Display: e = 0.06;c1 = [120 150 230]/255;c2 = ([120 150 230]+0)/383;c3 = ([120 150 230]+128)/383;patch([0 1 1 0],[0 0 1 1],c1);patch([0 1 1 1-e 1-e 0+e],[0 0 1 1-e 0+e 0+e],c2);patch([0 0 1 1-e 0+e 0+e],[0 1 1 1-e 1-e 0+e],c3);plot([0 1 1 0 0],[0 0 1 1 0]);disp('weights');
  "IW{2,1}(87,:)'" : Constant  Value=[0.75862055443656939;0.48151505598506017;0.39636866108651797;0.084938154926597481;-0.40332533459411019;0.62376381812181847;0.94471009830953523;0.42070184159691154;0.64430552551494635;0.88548776134268259]
      mask Display: e = 0.06;c1 = [120 150 230]/255;c2 = ([120 150 230]+0)/383;c3 = ([120 150 230]+128)/383;patch([0 1 1 0],[0 0 1 1],c1);patch([0 1 1 1-e 1-e 0+e],[0 0 1 1-e 0+e 0+e],c2);patch([0 0 1 1-e 0+e 0+e],[0 1 1 1-e 1-e 0+e],c3);plot([0 1 1 0 0],[0 0 1 1 0]);disp('weights');
  "IW{2,1}(88,:)'" : Constant  Value=[1.1427506826169753;0.62936587922505449;-0.49004829284384355;-0.46048001743492728;-0.021999420107764664;0.23291043008726525;-0.19183574261876263;0.017741740262746497;0.42680724909904078;-0.69481506039286023]
      mask Display: e = 0.06;c1 = [120 150 230]/255;c2 = ([120 150 230]+0)/383;c3 = ([120 150 230]+128)/383;patch([0 1 1 0],[0 0 1 1],c1);patch([0 1 1 1-e 1-e 0+e],[0 0 1 1-e 0+e 0+e],c2);patch([0 0 1 1-e 0+e 0+e],[0 1 1 1-e 1-e 0+e],c3);plot([0 1 1 0 0],[0 0 1 1 0]);disp('weights');
  "IW{2,1}(89,:)'" : Constant  Value=[0.94910616216646093;0.41058070107971867;0.62529909273938777;-0.3011703097552112;0.3972078522931129;-0.02577128685026242;0.017299420719741693;-0.0034381628090092431;0.47351107935826758;-0.77736700872214437]
      mask Display: e = 0.06;c1 = [120 150 230]/255;c2 = ([120 150 230]+0)/383;c3 = ([120 150 230]+128)/383;patch([0 1 1 0],[0 0 1 1],c1);patch([0 1 1 1-e 1-e 0+e],[0 0 1 1-e 0+e 0+e],c2);patch([0 0 1 1-e 0+e 0+e],[0 1 1 1-e 1-e 0+e],c3);plot([0 1 1 0 0],[0 0 1 1 0]);disp('weights');
  "IW{2,1}(9,:)'" : Constant  Value=[1.0160796294573236;0.59269011345627154;0.63894970976973076;-0.28237090002933934;-0.33124924843555648;-0.04315456757563102;-0.68282667032890232;-0.46324680507088412;0.99444413299782086;-0.81089233090211743]
      mask Display: e = 0.06;c1 = [120 150 230]/255;c2 = ([120 150 230]+0)/383;c3 = ([120 150 230]+128)/383;patch([0 1 1 0],[0 0 1 1],c1);patch([0 1 1 1-e 1-e 0+e],[0 0 1 1-e 0+e 0+e],c2);patch([0 0 1 1-e 0+e 0+e],[0 1 1 1-e 1-e 0+e],c3);plot([0 1 1 0 0],[0 0 1 1 0]);disp('weights');
  "IW{2,1}(90,:)'" : Constant  Value=[0.46215489347333705;-0.84365259680709581;-0.79455837508012572;-0.252742377507295;0.13703541465012928;0.22809504410599046;0.54277310506191112;0.44347872424620616;0.84730363427071254;-0.70460122308212525]
      mask Display: e = 0.06;c1 = [120 150 230]/255;c2 = ([120 150 230]+0)/383;c3 = ([120 150 230]+128)/383;patch([0 1 1 0],[0 0 1 1],c1);patch([0 1 1 1-e 1-e 0+e],[0 0 1 1-e 0+e 0+e],c2);patch([0 0 1 1-e 0+e 0+e],[0 1 1 1-e 1-e 0+e],c3);plot([0 1 1 0 0],[0 0 1 1 0]);disp('weights');
  "IW{2,1}(91,:)'" : Constant  Value=[0.96795348782537749;-0.77923874645364921;0.24975069605344119;0.58289120444432507;0.74228163187040819;-0.24322105584028259;-0.46790613338574527;0.56378406439285766;1.0152292394094584;0.34204584972294905]
      mask Display: e = 0.06;c1 = [120 150 230]/255;c2 = ([120 150 230]+0)/383;c3 = ([120 150 230]+128)/383;patch([0 1 1 0],[0 0 1 1],c1);patch([0 1 1 1-e 1-e 0+e],[0 0 1 1-e 0+e 0+e],c2);patch([0 0 1 1-e 0+e 0+e],[0 1 1 1-e 1-e 0+e],c3);plot([0 1 1 0 0],[0 0 1 1 0]);disp('weights');
  "IW{2,1}(92,:)'" : Constant  Value=[1.0347208187370875;-0.20027526312165078;-0.54796645613289929;0.0068518569790810835;0.13823489930375371;0.0074309428297270053;0.13642913228073272;0.39900093686247617;-0.59136236543321685;-0.8568417221654947]
      mask Display: e = 0.06;c1 = [120 150 230]/255;c2 = ([120 150 230]+0)/383;c3 = ([120 150 230]+128)/383;patch([0 1 1 0],[0 0 1 1],c1);patch([0 1 1 1-e 1-e 0+e],[0 0 1 1-e 0+e 0+e],c2);patch([0 0 1 1-e 0+e 0+e],[0 1 1 1-e 1-e 0+e],c3);plot([0 1 1 0 0],[0 0 1 1 0]);disp('weights');
  "IW{2,1}(93,:)'" : Constant  Value=[-0.18835327180921915;-0.52562189585372499;0.95622014193169469;-0.58720032303091607;1.065786212130913;0.21851205331429757;0.42526927252632141;0.44199791009720801;1.0014177164928308;-0.36317390585806236]
      mask Display: e = 0.06;c1 = [120 150 230]/255;c2 = ([120 150 230]+0)/383;c3 = ([120 150 230]+128)/383;patch([0 1 1 0],[0 0 1 1],c1);patch([0 1 1 1-e 1-e 0+e],[0 0 1 1-e 0+e 0+e],c2);patch([0 0 1 1-e 0+e 0+e],[0 1 1 1-e 1-e 0+e],c3);plot([0 1 1 0 0],[0 0 1 1 0]);disp('weights');
  "IW{2,1}(94,:)'" : Constant  Value=[0.36062921946687676;-0.10296675570248211;0.28594243972123434;-0.3992071133270042;0.707833203710026;0.16981939672380703;0.42057275496590252;0.18798154327821676;0.53105225417609214;0.065644044376200694]
      mask Display: e = 0.06;c1 = [120 150 230]/255;c2 = ([120 150 230]+0)/383;c3 = ([120 150 230]+128)/383;patch([0 1 1 0],[0 0 1 1],c1);patch([0 1 1 1-e 1-e 0+e],[0 0 1 1-e 0+e 0+e],c2);patch([0 0 1 1-e 0+e 0+e],[0 1 1 1-e 1-e 0+e],c3);plot([0 1 1 0 0],[0 0 1 1 0]);disp('weights');
  "IW{2,1}(95,:)'" : Constant  Value=[0.87318556352258292;-0.28264594987575059;-0.19144144360633808;0.43790753201637261;0.095554464908614967;0.5421098584585482;-0.22977759513649057;0.45241120459928819;-0.40201335825391704;0.06908732445909066]
      mask Display: e = 0.06;c1 = [120 150 230]/255;c2 = ([120 150 230]+0)/383;c3 = ([120 150 230]+128)/383;patch([0 1 1 0],[0 0 1 1],c1);patch([0 1 1 1-e 1-e 0+e],[0 0 1 1-e 0+e 0+e],c2);patch([0 0 1 1-e 0+e 0+e],[0 1 1 1-e 1-e 0+e],c3);plot([0 1 1 0 0],[0 0 1 1 0]);disp('weights');
  "IW{2,1}(96,:)'" : Constant  Value=[0.13471987067022076;0.57446780053583391;-0.29970722906873293;-0.54114299338516381;-0.71805525765441003;0.3463476503878089;-0.95402009501131801;-0.55142739799361484;0.25137287089026622;0.39159084740343381]
      mask Display: e = 0.06;c1 = [120 150 230]/255;c2 = ([120 150 230]+0)/383;c3 = ([120 150 230]+128)/383;patch([0 1 1 0],[0 0 1 1],c1);patch([0 1 1 1-e 1-e 0+e],[0 0 1 1-e 0+e 0+e],c2);patch([0 0 1 1-e 0+e 0+e],[0 1 1 1-e 1-e 0+e],c3);plot([0 1 1 0 0],[0 0 1 1 0]);disp('weights');
  "IW{2,1}(97,:)'" : Constant  Value=[-0.066949230085976266;0.31144443058415938;0.28955980814251281;-0.54624814446359349;0.77754163925464481;0.26824709385778606;0.43474713770048234;0.7564263278403196;0.83939170514915362;-0.00090188884432507166]
      mask Display: e = 0.06;c1 = [120 150 230]/255;c2 = ([120 150 230]+0)/383;c3 = ([120 150 230]+128)/383;patch([0 1 1 0],[0 0 1 1],c1);patch([0 1 1 1-e 1-e 0+e],[0 0 1 1-e 0+e 0+e],c2);patch([0 0 1 1-e 0+e 0+e],[0 1 1 1-e 1-e 0+e],c3);plot([0 1 1 0 0],[0 0 1 1 0]);disp('weights');
  "IW{2,1}(98,:)'" : Constant  Value=[0.23695028018267936;0.21782579182305323;-0.4283259664020212;0.18426537199475396;1.2566450258212249;0.3568321759413513;0.56600247721081387;-0.19602551881540314;0.72596897822143847;0.14395972887886688]
      mask Display: e = 0.06;c1 = [120 150 230]/255;c2 = ([120 150 230]+0)/383;c3 = ([120 150 230]+128)/383;patch([0 1 1 0],[0 0 1 1],c1);patch([0 1 1 1-e 1-e 0+e],[0 0 1 1-e 0+e 0+e],c2);patch([0 0 1 1-e 0+e 0+e],[0 1 1 1-e 1-e 0+e],c3);plot([0 1 1 0 0],[0 0 1 1 0]);disp('weights');
  "IW{2,1}(99,:)'" : Constant  Value=[-0.33201793504328031;0.50046304790390272;-1.2443681910239732;-0.70170257394515057;1.1942739623540282;0.66471097074503427;0.28460497036519461;-0.41447620098434101;0.77690762431157978;0.44384419183494772]
      mask Display: e = 0.06;c1 = [120 150 230]/255;c2 = ([120 150 230]+0)/383;c3 = ([120 150 230]+128)/383;patch([0 1 1 0],[0 0 1 1],c1);patch([0 1 1 1-e 1-e 0+e],[0 0 1 1-e 0+e 0+e],c2);patch([0 0 1 1-e 0+e 0+e],[0 1 1 1-e 1-e 0+e],c3);plot([0 1 1 0 0],[0 0 1 1 0]);disp('weights');
  Mux : Mux  Inputs=405
      mask Display: e = 0.06;c1 = [120 150 230]/255;c2 = ([120 150 230]+0)/383;c3 = ([120 150 230]+128)/383;patch([0 1 1 0],[0 0 1 1],c1);patch([0 1 1 1-e 1-e 0+e],[0 0 1 1-e 0+e 0+e],c2);patch([0 0 1 1-e 0+e 0+e],[0 1 1 1-e 1-e 0+e],c3);plot([0 1 1 0 0],[0 0 1 1 0]);disp('Mux');
  dotprod{1..405} (405 alike) : neural/Weight Functions/dotprod
  "lz{2,1}" : Outport
      mask Display: e = 0.06;c1 = [120 230 180]/255;c2 = ([120 230 180]+0)/(256+128);c3 = ([120 230 180]+128)/(256+128);patch([0 1 1 0],[0 0 1 1],c1);patch([0 1 1 1-e 1-e 0+e],[0 0 1 1-e 0+e 0+e],c2);patch([0 0 1 1-e 0+e 0+e],[0 1 1 1-e 1-e 0+e],c3);plot([0 1 1 0 0],[0 0 1 1 0]);
  wires:
  "IW{2,1}(1,:)'"/1 -> dotprod1/1
  "ad{2,1}"/1 -> dotprod1/2, dotprod2/2, dotprod3/2, dotprod4/2, dotprod5/2, dotprod6/2, dotprod7/2, dotprod8/2, dotprod9/2, dotprod10/2, dotprod11/2, dotprod12/2, dotprod13/2, dotprod14/2, dotprod15/2, dotprod16/2, dotprod17/2, dotprod18/2, dotprod19/2, dotprod20/2, dotprod21/2, dotprod22/2, dotprod23/2, dotprod24/2, dotprod25/2, dotprod26/2, dotprod27/2, dotprod28/2, dotprod29/2, dotprod30/2, dotprod31/2, dotprod32/2, dotprod33/2, dotprod34/2, dotprod35/2, dotprod36/2, dotprod37/2, dotprod38/2, dotprod39/2, dotprod40/2, dotprod41/2, dotprod42/2, dotprod43/2, dotprod44/2, dotprod45/2, dotprod46/2, dotprod47/2, dotprod48/2, dotprod49/2, dotprod50/2, dotprod51/2, dotprod52/2, dotprod53/2, dotprod54/2, dotprod55/2, dotprod56/2, dotprod57/2, dotprod58/2, dotprod59/2, dotprod60/2, dotprod61/2, dotprod62/2, dotprod63/2, dotprod64/2, dotprod65/2, dotprod66/2, dotprod67/2, dotprod68/2, dotprod69/2, dotprod70/2, dotprod71/2, dotprod72/2, dotprod73/2, dotprod74/2, dotprod75/2, dotprod76/2, dotprod77/2, dotprod78/2, dotprod79/2, dotprod80/2, dotprod81/2, dotprod82/2, dotprod83/2, dotprod84/2, dotprod85/2, dotprod86/2, dotprod87/2, dotprod88/2, dotprod89/2, dotprod90/2, dotprod91/2, dotprod92/2, dotprod93/2, dotprod94/2, dotprod95/2, dotprod96/2, dotprod97/2, dotprod98/2, dotprod99/2, dotprod100/2, dotprod101/2, dotprod102/2, dotprod103/2, dotprod104/2, dotprod105/2, dotprod106/2, dotprod107/2, dotprod108/2, dotprod109/2, dotprod110/2, dotprod111/2, dotprod112/2, dotprod113/2, dotprod114/2, dotprod115/2, dotprod116/2, dotprod117/2, dotprod118/2, dotprod119/2, dotprod120/2, dotprod121/2, dotprod122/2, dotprod123/2, dotprod124/2, dotprod125/2, dotprod126/2, dotprod127/2, dotprod128/2, dotprod129/2, dotprod130/2, dotprod131/2, dotprod132/2, dotprod133/2, dotprod134/2, dotprod135/2, dotprod136/2, dotprod137/2, dotprod138/2, dotprod139/2, dotprod140/2, dotprod141/2, dotprod142/2, dotprod143/2, dotprod144/2, dotprod145/2, dotprod146/2, dotprod147/2, dotprod148/2, dotprod149/2, dotprod150/2, dotprod151/2, dotprod152/2, dotprod153/2, dotprod154/2, dotprod155/2, dotprod156/2, dotprod157/2, dotprod158/2, dotprod159/2, dotprod160/2, dotprod161/2, dotprod162/2, dotprod163/2, dotprod164/2, dotprod165/2, dotprod166/2, dotprod167/2, dotprod168/2, dotprod169/2, dotprod170/2, dotprod171/2, dotprod172/2, dotprod173/2, dotprod174/2, dotprod175/2, dotprod176/2, dotprod177/2, dotprod178/2, dotprod179/2, dotprod180/2, dotprod181/2, dotprod182/2, dotprod183/2, dotprod184/2, dotprod185/2, dotprod186/2, dotprod187/2, dotprod188/2, dotprod189/2, dotprod190/2, dotprod191/2, dotprod192/2, dotprod193/2, dotprod194/2, dotprod195/2, dotprod196/2, dotprod197/2, dotprod198/2, dotprod199/2, dotprod200/2, dotprod201/2, dotprod202/2, dotprod203/2, dotprod204/2, dotprod205/2, dotprod206/2, dotprod207/2, dotprod208/2, dotprod209/2, dotprod210/2, dotprod211/2, dotprod212/2, dotprod213/2, dotprod214/2, dotprod215/2, dotprod216/2, dotprod217/2, dotprod218/2, dotprod219/2, dotprod220/2, dotprod221/2, dotprod222/2, dotprod223/2, dotprod224/2, dotprod225/2, dotprod226/2, dotprod227/2, dotprod228/2, dotprod229/2, dotprod230/2, dotprod231/2, dotprod232/2, dotprod233/2, dotprod234/2, dotprod235/2, dotprod236/2, dotprod237/2, dotprod238/2, dotprod239/2, dotprod240/2, dotprod241/2, dotprod242/2, dotprod243/2, dotprod244/2, dotprod245/2, dotprod246/2, dotprod247/2, dotprod248/2, dotprod249/2, dotprod250/2, dotprod251/2, dotprod252/2, dotprod253/2, dotprod254/2, dotprod255/2, dotprod256/2, dotprod257/2, dotprod258/2, dotprod259/2, dotprod260/2, dotprod261/2, dotprod262/2, dotprod263/2, dotprod264/2, dotprod265/2, dotprod266/2, dotprod267/2, dotprod268/2, dotprod269/2, dotprod270/2, dotprod271/2, dotprod272/2, dotprod273/2, dotprod274/2, dotprod275/2, dotprod276/2, dotprod277/2, dotprod278/2, dotprod279/2, dotprod280/2, dotprod281/2, dotprod282/2, dotprod283/2, dotprod284/2, dotprod285/2, dotprod286/2, dotprod287/2, dotprod288/2, dotprod289/2, dotprod290/2, dotprod291/2, dotprod292/2, dotprod293/2, dotprod294/2, dotprod295/2, dotprod296/2, dotprod297/2, dotprod298/2, dotprod299/2, dotprod300/2, dotprod301/2, dotprod302/2, dotprod303/2, dotprod304/2, dotprod305/2, dotprod306/2, dotprod307/2, dotprod308/2, dotprod309/2, dotprod310/2, dotprod311/2, dotprod312/2, dotprod313/2, dotprod314/2, dotprod315/2, dotprod316/2, dotprod317/2, dotprod318/2, dotprod319/2, dotprod320/2, dotprod321/2, dotprod322/2, dotprod323/2, dotprod324/2, dotprod325/2, dotprod326/2, dotprod327/2, dotprod328/2, dotprod329/2, dotprod330/2, dotprod331/2, dotprod332/2, dotprod333/2, dotprod334/2, dotprod335/2, dotprod336/2, dotprod337/2, dotprod338/2, dotprod339/2, dotprod340/2, dotprod341/2, dotprod342/2, dotprod343/2, dotprod344/2, dotprod345/2, dotprod346/2, dotprod347/2, dotprod348/2, dotprod349/2, dotprod350/2, dotprod351/2, dotprod352/2, dotprod353/2, dotprod354/2, dotprod355/2, dotprod356/2, dotprod357/2, dotprod358/2, dotprod359/2, dotprod360/2, dotprod361/2, dotprod362/2, dotprod363/2, dotprod364/2, dotprod365/2, dotprod366/2, dotprod367/2, dotprod368/2, dotprod369/2, dotprod370/2, dotprod371/2, dotprod372/2, dotprod373/2, dotprod374/2, dotprod375/2, dotprod376/2, dotprod377/2, dotprod378/2, dotprod379/2, dotprod380/2, dotprod381/2, dotprod382/2, dotprod383/2, dotprod384/2, dotprod385/2, dotprod386/2, dotprod387/2, dotprod388/2, dotprod389/2, dotprod390/2, dotprod391/2, dotprod392/2, dotprod393/2, dotprod394/2, dotprod395/2, dotprod396/2, dotprod397/2, dotprod398/2, dotprod399/2, dotprod400/2, dotprod401/2, dotprod402/2, dotprod403/2, dotprod404/2, dotprod405/2
  dotprod1/1 -> Mux/1
  "IW{2,1}(2,:)'"/1 -> dotprod2/1
  dotprod2/1 -> Mux/2
  "IW{2,1}(3,:)'"/1 -> dotprod3/1
  dotprod3/1 -> Mux/3
  "IW{2,1}(4,:)'"/1 -> dotprod4/1
  dotprod4/1 -> Mux/4
  "IW{2,1}(5,:)'"/1 -> dotprod5/1
  dotprod5/1 -> Mux/5
  "IW{2,1}(6,:)'"/1 -> dotprod6/1
  dotprod6/1 -> Mux/6
  "IW{2,1}(7,:)'"/1 -> dotprod7/1
  dotprod7/1 -> Mux/7
  "IW{2,1}(8,:)'"/1 -> dotprod8/1
  dotprod8/1 -> Mux/8
  "IW{2,1}(9,:)'"/1 -> dotprod9/1
  dotprod9/1 -> Mux/9
  "IW{2,1}(10,:)'"/1 -> dotprod10/1
  dotprod10/1 -> Mux/10
  "IW{2,1}(11,:)'"/1 -> dotprod11/1
  dotprod11/1 -> Mux/11
  "IW{2,1}(12,:)'"/1 -> dotprod12/1
  dotprod12/1 -> Mux/12
  "IW{2,1}(13,:)'"/1 -> dotprod13/1
  dotprod13/1 -> Mux/13
  "IW{2,1}(14,:)'"/1 -> dotprod14/1
  dotprod14/1 -> Mux/14
  "IW{2,1}(15,:)'"/1 -> dotprod15/1
  dotprod15/1 -> Mux/15
  "IW{2,1}(16,:)'"/1 -> dotprod16/1
  dotprod16/1 -> Mux/16
  "IW{2,1}(17,:)'"/1 -> dotprod17/1
  dotprod17/1 -> Mux/17
  "IW{2,1}(18,:)'"/1 -> dotprod18/1
  dotprod18/1 -> Mux/18
  "IW{2,1}(19,:)'"/1 -> dotprod19/1
  dotprod19/1 -> Mux/19
  "IW{2,1}(20,:)'"/1 -> dotprod20/1
  dotprod20/1 -> Mux/20
  "IW{2,1}(21,:)'"/1 -> dotprod21/1
  dotprod21/1 -> Mux/21
  "IW{2,1}(22,:)'"/1 -> dotprod22/1
  dotprod22/1 -> Mux/22
  "IW{2,1}(23,:)'"/1 -> dotprod23/1
  dotprod23/1 -> Mux/23
  "IW{2,1}(24,:)'"/1 -> dotprod24/1
  dotprod24/1 -> Mux/24
  "IW{2,1}(25,:)'"/1 -> dotprod25/1
  dotprod25/1 -> Mux/25
  "IW{2,1}(26,:)'"/1 -> dotprod26/1
  dotprod26/1 -> Mux/26
  "IW{2,1}(27,:)'"/1 -> dotprod27/1
  dotprod27/1 -> Mux/27
  "IW{2,1}(28,:)'"/1 -> dotprod28/1
  dotprod28/1 -> Mux/28
  "IW{2,1}(29,:)'"/1 -> dotprod29/1
  dotprod29/1 -> Mux/29
  "IW{2,1}(30,:)'"/1 -> dotprod30/1
  dotprod30/1 -> Mux/30
  "IW{2,1}(31,:)'"/1 -> dotprod31/1
  dotprod31/1 -> Mux/31
  "IW{2,1}(32,:)'"/1 -> dotprod32/1
  dotprod32/1 -> Mux/32
  "IW{2,1}(33,:)'"/1 -> dotprod33/1
  dotprod33/1 -> Mux/33
  "IW{2,1}(34,:)'"/1 -> dotprod34/1
  dotprod34/1 -> Mux/34
  "IW{2,1}(35,:)'"/1 -> dotprod35/1
  dotprod35/1 -> Mux/35
  "IW{2,1}(36,:)'"/1 -> dotprod36/1
  dotprod36/1 -> Mux/36
  "IW{2,1}(37,:)'"/1 -> dotprod37/1
  dotprod37/1 -> Mux/37
  "IW{2,1}(38,:)'"/1 -> dotprod38/1
  dotprod38/1 -> Mux/38
  "IW{2,1}(39,:)'"/1 -> dotprod39/1
  dotprod39/1 -> Mux/39
  "IW{2,1}(40,:)'"/1 -> dotprod40/1
  dotprod40/1 -> Mux/40
  "IW{2,1}(41,:)'"/1 -> dotprod41/1
  dotprod41/1 -> Mux/41
  "IW{2,1}(42,:)'"/1 -> dotprod42/1
  dotprod42/1 -> Mux/42
  "IW{2,1}(43,:)'"/1 -> dotprod43/1
  dotprod43/1 -> Mux/43
  "IW{2,1}(44,:)'"/1 -> dotprod44/1
  dotprod44/1 -> Mux/44
  "IW{2,1}(45,:)'"/1 -> dotprod45/1
  dotprod45/1 -> Mux/45
  "IW{2,1}(46,:)'"/1 -> dotprod46/1
  dotprod46/1 -> Mux/46
  "IW{2,1}(47,:)'"/1 -> dotprod47/1
  dotprod47/1 -> Mux/47
  "IW{2,1}(48,:)'"/1 -> dotprod48/1
  dotprod48/1 -> Mux/48
  "IW{2,1}(49,:)'"/1 -> dotprod49/1
  dotprod49/1 -> Mux/49
  "IW{2,1}(50,:)'"/1 -> dotprod50/1
  dotprod50/1 -> Mux/50
  "IW{2,1}(51,:)'"/1 -> dotprod51/1
  dotprod51/1 -> Mux/51
  "IW{2,1}(52,:)'"/1 -> dotprod52/1
  dotprod52/1 -> Mux/52
  "IW{2,1}(53,:)'"/1 -> dotprod53/1
  dotprod53/1 -> Mux/53
  "IW{2,1}(54,:)'"/1 -> dotprod54/1
  dotprod54/1 -> Mux/54
  "IW{2,1}(55,:)'"/1 -> dotprod55/1
  dotprod55/1 -> Mux/55
  "IW{2,1}(56,:)'"/1 -> dotprod56/1
  dotprod56/1 -> Mux/56
  "IW{2,1}(57,:)'"/1 -> dotprod57/1
  dotprod57/1 -> Mux/57
  "IW{2,1}(58,:)'"/1 -> dotprod58/1
  dotprod58/1 -> Mux/58
  "IW{2,1}(59,:)'"/1 -> dotprod59/1
  dotprod59/1 -> Mux/59
  "IW{2,1}(60,:)'"/1 -> dotprod60/1
  dotprod60/1 -> Mux/60
  "IW{2,1}(61,:)'"/1 -> dotprod61/1
  dotprod61/1 -> Mux/61
  "IW{2,1}(62,:)'"/1 -> dotprod62/1
  dotprod62/1 -> Mux/62
  "IW{2,1}(63,:)'"/1 -> dotprod63/1
  dotprod63/1 -> Mux/63
  "IW{2,1}(64,:)'"/1 -> dotprod64/1
  dotprod64/1 -> Mux/64
  "IW{2,1}(65,:)'"/1 -> dotprod65/1
  dotprod65/1 -> Mux/65
  "IW{2,1}(66,:)'"/1 -> dotprod66/1
  dotprod66/1 -> Mux/66
  "IW{2,1}(67,:)'"/1 -> dotprod67/1
  dotprod67/1 -> Mux/67
  "IW{2,1}(68,:)'"/1 -> dotprod68/1
  dotprod68/1 -> Mux/68
  "IW{2,1}(69,:)'"/1 -> dotprod69/1
  dotprod69/1 -> Mux/69
  "IW{2,1}(70,:)'"/1 -> dotprod70/1
  dotprod70/1 -> Mux/70
  "IW{2,1}(71,:)'"/1 -> dotprod71/1
  dotprod71/1 -> Mux/71
  "IW{2,1}(72,:)'"/1 -> dotprod72/1
  dotprod72/1 -> Mux/72
  "IW{2,1}(73,:)'"/1 -> dotprod73/1
  dotprod73/1 -> Mux/73
  "IW{2,1}(74,:)'"/1 -> dotprod74/1
  dotprod74/1 -> Mux/74
  "IW{2,1}(75,:)'"/1 -> dotprod75/1
  dotprod75/1 -> Mux/75
  "IW{2,1}(76,:)'"/1 -> dotprod76/1
  dotprod76/1 -> Mux/76
  "IW{2,1}(77,:)'"/1 -> dotprod77/1
  dotprod77/1 -> Mux/77
  "IW{2,1}(78,:)'"/1 -> dotprod78/1
  dotprod78/1 -> Mux/78
  "IW{2,1}(79,:)'"/1 -> dotprod79/1
  dotprod79/1 -> Mux/79
  "IW{2,1}(80,:)'"/1 -> dotprod80/1
  dotprod80/1 -> Mux/80
  "IW{2,1}(81,:)'"/1 -> dotprod81/1
  dotprod81/1 -> Mux/81
  "IW{2,1}(82,:)'"/1 -> dotprod82/1
  dotprod82/1 -> Mux/82
  "IW{2,1}(83,:)'"/1 -> dotprod83/1
  dotprod83/1 -> Mux/83
  "IW{2,1}(84,:)'"/1 -> dotprod84/1
  dotprod84/1 -> Mux/84
  "IW{2,1}(85,:)'"/1 -> dotprod85/1
  dotprod85/1 -> Mux/85
  "IW{2,1}(86,:)'"/1 -> dotprod86/1
  dotprod86/1 -> Mux/86
  "IW{2,1}(87,:)'"/1 -> dotprod87/1
  dotprod87/1 -> Mux/87
  "IW{2,1}(88,:)'"/1 -> dotprod88/1
  dotprod88/1 -> Mux/88
  "IW{2,1}(89,:)'"/1 -> dotprod89/1
  dotprod89/1 -> Mux/89
  "IW{2,1}(90,:)'"/1 -> dotprod90/1
  dotprod90/1 -> Mux/90
  "IW{2,1}(91,:)'"/1 -> dotprod91/1
  dotprod91/1 -> Mux/91
  "IW{2,1}(92,:)'"/1 -> dotprod92/1
  dotprod92/1 -> Mux/92
  "IW{2,1}(93,:)'"/1 -> dotprod93/1
  dotprod93/1 -> Mux/93
  "IW{2,1}(94,:)'"/1 -> dotprod94/1
  dotprod94/1 -> Mux/94
  "IW{2,1}(95,:)'"/1 -> dotprod95/1
  dotprod95/1 -> Mux/95
  "IW{2,1}(96,:)'"/1 -> dotprod96/1
  dotprod96/1 -> Mux/96
  "IW{2,1}(97,:)'"/1 -> dotprod97/1
  dotprod97/1 -> Mux/97
  "IW{2,1}(98,:)'"/1 -> dotprod98/1
  dotprod98/1 -> Mux/98
  "IW{2,1}(99,:)'"/1 -> dotprod99/1
  dotprod99/1 -> Mux/99
  "IW{2,1}(100,:)'"/1 -> dotprod100/1
  dotprod100/1 -> Mux/100
  "IW{2,1}(101,:)'"/1 -> dotprod101/1
  dotprod101/1 -> Mux/101
  "IW{2,1}(102,:)'"/1 -> dotprod102/1
  dotprod102/1 -> Mux/102
  "IW{2,1}(103,:)'"/1 -> dotprod103/1
  dotprod103/1 -> Mux/103
  "IW{2,1}(104,:)'"/1 -> dotprod104/1
  dotprod104/1 -> Mux/104
  "IW{2,1}(105,:)'"/1 -> dotprod105/1
  dotprod105/1 -> Mux/105
  "IW{2,1}(106,:)'"/1 -> dotprod106/1
  dotprod106/1 -> Mux/106
  "IW{2,1}(107,:)'"/1 -> dotprod107/1
  dotprod107/1 -> Mux/107
  "IW{2,1}(108,:)'"/1 -> dotprod108/1
  dotprod108/1 -> Mux/108
  "IW{2,1}(109,:)'"/1 -> dotprod109/1
  dotprod109/1 -> Mux/109
  "IW{2,1}(110,:)'"/1 -> dotprod110/1
  dotprod110/1 -> Mux/110
  "IW{2,1}(111,:)'"/1 -> dotprod111/1
  dotprod111/1 -> Mux/111
  "IW{2,1}(112,:)'"/1 -> dotprod112/1
  dotprod112/1 -> Mux/112
  "IW{2,1}(113,:)'"/1 -> dotprod113/1
  dotprod113/1 -> Mux/113
  "IW{2,1}(114,:)'"/1 -> dotprod114/1
  dotprod114/1 -> Mux/114
  "IW{2,1}(115,:)'"/1 -> dotprod115/1
  dotprod115/1 -> Mux/115
  "IW{2,1}(116,:)'"/1 -> dotprod116/1
  dotprod116/1 -> Mux/116
  "IW{2,1}(117,:)'"/1 -> dotprod117/1
  dotprod117/1 -> Mux/117
  "IW{2,1}(118,:)'"/1 -> dotprod118/1
  dotprod118/1 -> Mux/118
  "IW{2,1}(119,:)'"/1 -> dotprod119/1
  dotprod119/1 -> Mux/119
  "IW{2,1}(120,:)'"/1 -> dotprod120/1
  dotprod120/1 -> Mux/120
  "IW{2,1}(121,:)'"/1 -> dotprod121/1
  dotprod121/1 -> Mux/121
  "IW{2,1}(122,:)'"/1 -> dotprod122/1
  dotprod122/1 -> Mux/122
  "IW{2,1}(123,:)'"/1 -> dotprod123/1
  dotprod123/1 -> Mux/123
  "IW{2,1}(124,:)'"/1 -> dotprod124/1
  dotprod124/1 -> Mux/124
  "IW{2,1}(125,:)'"/1 -> dotprod125/1
  dotprod125/1 -> Mux/125
  "IW{2,1}(126,:)'"/1 -> dotprod126/1
  dotprod126/1 -> Mux/126
  "IW{2,1}(127,:)'"/1 -> dotprod127/1
  dotprod127/1 -> Mux/127
  "IW{2,1}(128,:)'"/1 -> dotprod128/1
  dotprod128/1 -> Mux/128
  "IW{2,1}(129,:)'"/1 -> dotprod129/1
  dotprod129/1 -> Mux/129
  "IW{2,1}(130,:)'"/1 -> dotprod130/1
  dotprod130/1 -> Mux/130
  "IW{2,1}(131,:)'"/1 -> dotprod131/1
  dotprod131/1 -> Mux/131
  "IW{2,1}(132,:)'"/1 -> dotprod132/1
  dotprod132/1 -> Mux/132
  "IW{2,1}(133,:)'"/1 -> dotprod133/1
  dotprod133/1 -> Mux/133
  "IW{2,1}(134,:)'"/1 -> dotprod134/1
  dotprod134/1 -> Mux/134
  "IW{2,1}(135,:)'"/1 -> dotprod135/1
  dotprod135/1 -> Mux/135
  "IW{2,1}(136,:)'"/1 -> dotprod136/1
  dotprod136/1 -> Mux/136
  "IW{2,1}(137,:)'"/1 -> dotprod137/1
  dotprod137/1 -> Mux/137
  "IW{2,1}(138,:)'"/1 -> dotprod138/1
  dotprod138/1 -> Mux/138
  "IW{2,1}(139,:)'"/1 -> dotprod139/1
  dotprod139/1 -> Mux/139
  "IW{2,1}(140,:)'"/1 -> dotprod140/1
  dotprod140/1 -> Mux/140
  "IW{2,1}(141,:)'"/1 -> dotprod141/1
  dotprod141/1 -> Mux/141
  "IW{2,1}(142,:)'"/1 -> dotprod142/1
  dotprod142/1 -> Mux/142
  "IW{2,1}(143,:)'"/1 -> dotprod143/1
  dotprod143/1 -> Mux/143
  "IW{2,1}(144,:)'"/1 -> dotprod144/1
  dotprod144/1 -> Mux/144
  "IW{2,1}(145,:)'"/1 -> dotprod145/1
  dotprod145/1 -> Mux/145
  "IW{2,1}(146,:)'"/1 -> dotprod146/1
  dotprod146/1 -> Mux/146
  "IW{2,1}(147,:)'"/1 -> dotprod147/1
  dotprod147/1 -> Mux/147
  "IW{2,1}(148,:)'"/1 -> dotprod148/1
  dotprod148/1 -> Mux/148
  "IW{2,1}(149,:)'"/1 -> dotprod149/1
  dotprod149/1 -> Mux/149
  "IW{2,1}(150,:)'"/1 -> dotprod150/1
  dotprod150/1 -> Mux/150
  "IW{2,1}(151,:)'"/1 -> dotprod151/1
  dotprod151/1 -> Mux/151
  "IW{2,1}(152,:)'"/1 -> dotprod152/1
  dotprod152/1 -> Mux/152
  "IW{2,1}(153,:)'"/1 -> dotprod153/1
  dotprod153/1 -> Mux/153
  "IW{2,1}(154,:)'"/1 -> dotprod154/1
  dotprod154/1 -> Mux/154
  "IW{2,1}(155,:)'"/1 -> dotprod155/1
  dotprod155/1 -> Mux/155
  "IW{2,1}(156,:)'"/1 -> dotprod156/1
  dotprod156/1 -> Mux/156
  "IW{2,1}(157,:)'"/1 -> dotprod157/1
  dotprod157/1 -> Mux/157
  "IW{2,1}(158,:)'"/1 -> dotprod158/1
  dotprod158/1 -> Mux/158
  "IW{2,1}(159,:)'"/1 -> dotprod159/1
  dotprod159/1 -> Mux/159
  "IW{2,1}(160,:)'"/1 -> dotprod160/1
  dotprod160/1 -> Mux/160
  "IW{2,1}(161,:)'"/1 -> dotprod161/1
  dotprod161/1 -> Mux/161
  "IW{2,1}(162,:)'"/1 -> dotprod162/1
  dotprod162/1 -> Mux/162
  "IW{2,1}(163,:)'"/1 -> dotprod163/1
  dotprod163/1 -> Mux/163
  "IW{2,1}(164,:)'"/1 -> dotprod164/1
  dotprod164/1 -> Mux/164
  "IW{2,1}(165,:)'"/1 -> dotprod165/1
  dotprod165/1 -> Mux/165
  "IW{2,1}(166,:)'"/1 -> dotprod166/1
  dotprod166/1 -> Mux/166
  "IW{2,1}(167,:)'"/1 -> dotprod167/1
  dotprod167/1 -> Mux/167
  "IW{2,1}(168,:)'"/1 -> dotprod168/1
  dotprod168/1 -> Mux/168
  "IW{2,1}(169,:)'"/1 -> dotprod169/1
  dotprod169/1 -> Mux/169
  "IW{2,1}(170,:)'"/1 -> dotprod170/1
  dotprod170/1 -> Mux/170
  "IW{2,1}(171,:)'"/1 -> dotprod171/1
  dotprod171/1 -> Mux/171
  "IW{2,1}(172,:)'"/1 -> dotprod172/1
  dotprod172/1 -> Mux/172
  "IW{2,1}(173,:)'"/1 -> dotprod173/1
  dotprod173/1 -> Mux/173
  "IW{2,1}(174,:)'"/1 -> dotprod174/1
  dotprod174/1 -> Mux/174
  "IW{2,1}(175,:)'"/1 -> dotprod175/1
  dotprod175/1 -> Mux/175
  "IW{2,1}(176,:)'"/1 -> dotprod176/1
  dotprod176/1 -> Mux/176
  "IW{2,1}(177,:)'"/1 -> dotprod177/1
  dotprod177/1 -> Mux/177
  "IW{2,1}(178,:)'"/1 -> dotprod178/1
  dotprod178/1 -> Mux/178
  "IW{2,1}(179,:)'"/1 -> dotprod179/1
  dotprod179/1 -> Mux/179
  "IW{2,1}(180,:)'"/1 -> dotprod180/1
  dotprod180/1 -> Mux/180
  "IW{2,1}(181,:)'"/1 -> dotprod181/1
  dotprod181/1 -> Mux/181
  "IW{2,1}(182,:)'"/1 -> dotprod182/1
  dotprod182/1 -> Mux/182
  "IW{2,1}(183,:)'"/1 -> dotprod183/1
  dotprod183/1 -> Mux/183
  "IW{2,1}(184,:)'"/1 -> dotprod184/1
  dotprod184/1 -> Mux/184
  "IW{2,1}(185,:)'"/1 -> dotprod185/1
  dotprod185/1 -> Mux/185
  "IW{2,1}(186,:)'"/1 -> dotprod186/1
  dotprod186/1 -> Mux/186
  "IW{2,1}(187,:)'"/1 -> dotprod187/1
  dotprod187/1 -> Mux/187
  "IW{2,1}(188,:)'"/1 -> dotprod188/1
  dotprod188/1 -> Mux/188
  "IW{2,1}(189,:)'"/1 -> dotprod189/1
  dotprod189/1 -> Mux/189
  "IW{2,1}(190,:)'"/1 -> dotprod190/1
  dotprod190/1 -> Mux/190
  "IW{2,1}(191,:)'"/1 -> dotprod191/1
  dotprod191/1 -> Mux/191
  "IW{2,1}(192,:)'"/1 -> dotprod192/1
  dotprod192/1 -> Mux/192
  "IW{2,1}(193,:)'"/1 -> dotprod193/1
  dotprod193/1 -> Mux/193
  "IW{2,1}(194,:)'"/1 -> dotprod194/1
  dotprod194/1 -> Mux/194
  "IW{2,1}(195,:)'"/1 -> dotprod195/1
  dotprod195/1 -> Mux/195
  "IW{2,1}(196,:)'"/1 -> dotprod196/1
  dotprod196/1 -> Mux/196
  "IW{2,1}(197,:)'"/1 -> dotprod197/1
  dotprod197/1 -> Mux/197
  "IW{2,1}(198,:)'"/1 -> dotprod198/1
  dotprod198/1 -> Mux/198
  "IW{2,1}(199,:)'"/1 -> dotprod199/1
  dotprod199/1 -> Mux/199
  "IW{2,1}(200,:)'"/1 -> dotprod200/1
  dotprod200/1 -> Mux/200
  "IW{2,1}(201,:)'"/1 -> dotprod201/1
  dotprod201/1 -> Mux/201
  "IW{2,1}(202,:)'"/1 -> dotprod202/1
  dotprod202/1 -> Mux/202
  "IW{2,1}(203,:)'"/1 -> dotprod203/1
  dotprod203/1 -> Mux/203
  "IW{2,1}(204,:)'"/1 -> dotprod204/1
  dotprod204/1 -> Mux/204
  "IW{2,1}(205,:)'"/1 -> dotprod205/1
  dotprod205/1 -> Mux/205
  "IW{2,1}(206,:)'"/1 -> dotprod206/1
  dotprod206/1 -> Mux/206
  "IW{2,1}(207,:)'"/1 -> dotprod207/1
  dotprod207/1 -> Mux/207
  "IW{2,1}(208,:)'"/1 -> dotprod208/1
  dotprod208/1 -> Mux/208
  "IW{2,1}(209,:)'"/1 -> dotprod209/1
  dotprod209/1 -> Mux/209
  "IW{2,1}(210,:)'"/1 -> dotprod210/1
  dotprod210/1 -> Mux/210
  "IW{2,1}(211,:)'"/1 -> dotprod211/1
  dotprod211/1 -> Mux/211
  "IW{2,1}(212,:)'"/1 -> dotprod212/1
  dotprod212/1 -> Mux/212
  "IW{2,1}(213,:)'"/1 -> dotprod213/1
  dotprod213/1 -> Mux/213
  "IW{2,1}(214,:)'"/1 -> dotprod214/1
  dotprod214/1 -> Mux/214
  "IW{2,1}(215,:)'"/1 -> dotprod215/1
  dotprod215/1 -> Mux/215
  "IW{2,1}(216,:)'"/1 -> dotprod216/1
  dotprod216/1 -> Mux/216
  "IW{2,1}(217,:)'"/1 -> dotprod217/1
  dotprod217/1 -> Mux/217
  "IW{2,1}(218,:)'"/1 -> dotprod218/1
  dotprod218/1 -> Mux/218
  "IW{2,1}(219,:)'"/1 -> dotprod219/1
  dotprod219/1 -> Mux/219
  "IW{2,1}(220,:)'"/1 -> dotprod220/1
  dotprod220/1 -> Mux/220
  "IW{2,1}(221,:)'"/1 -> dotprod221/1
  dotprod221/1 -> Mux/221
  "IW{2,1}(222,:)'"/1 -> dotprod222/1
  dotprod222/1 -> Mux/222
  "IW{2,1}(223,:)'"/1 -> dotprod223/1
  dotprod223/1 -> Mux/223
  "IW{2,1}(224,:)'"/1 -> dotprod224/1
  dotprod224/1 -> Mux/224
  "IW{2,1}(225,:)'"/1 -> dotprod225/1
  dotprod225/1 -> Mux/225
  "IW{2,1}(226,:)'"/1 -> dotprod226/1
  dotprod226/1 -> Mux/226
  "IW{2,1}(227,:)'"/1 -> dotprod227/1
  dotprod227/1 -> Mux/227
  "IW{2,1}(228,:)'"/1 -> dotprod228/1
  dotprod228/1 -> Mux/228
  "IW{2,1}(229,:)'"/1 -> dotprod229/1
  dotprod229/1 -> Mux/229
  "IW{2,1}(230,:)'"/1 -> dotprod230/1
  dotprod230/1 -> Mux/230
  "IW{2,1}(231,:)'"/1 -> dotprod231/1
  dotprod231/1 -> Mux/231
  "IW{2,1}(232,:)'"/1 -> dotprod232/1
  dotprod232/1 -> Mux/232
  "IW{2,1}(233,:)'"/1 -> dotprod233/1
  dotprod233/1 -> Mux/233
  "IW{2,1}(234,:)'"/1 -> dotprod234/1
  dotprod234/1 -> Mux/234
  "IW{2,1}(235,:)'"/1 -> dotprod235/1
  dotprod235/1 -> Mux/235
  "IW{2,1}(236,:)'"/1 -> dotprod236/1
  dotprod236/1 -> Mux/236
  "IW{2,1}(237,:)'"/1 -> dotprod237/1
  dotprod237/1 -> Mux/237
  "IW{2,1}(238,:)'"/1 -> dotprod238/1
  dotprod238/1 -> Mux/238
  "IW{2,1}(239,:)'"/1 -> dotprod239/1
  dotprod239/1 -> Mux/239
  "IW{2,1}(240,:)'"/1 -> dotprod240/1
  dotprod240/1 -> Mux/240
  "IW{2,1}(241,:)'"/1 -> dotprod241/1
  dotprod241/1 -> Mux/241
  "IW{2,1}(242,:)'"/1 -> dotprod242/1
  dotprod242/1 -> Mux/242
  "IW{2,1}(243,:)'"/1 -> dotprod243/1
  dotprod243/1 -> Mux/243
  "IW{2,1}(244,:)'"/1 -> dotprod244/1
  dotprod244/1 -> Mux/244
  "IW{2,1}(245,:)'"/1 -> dotprod245/1
  dotprod245/1 -> Mux/245
  "IW{2,1}(246,:)'"/1 -> dotprod246/1
  dotprod246/1 -> Mux/246
  "IW{2,1}(247,:)'"/1 -> dotprod247/1
  dotprod247/1 -> Mux/247
  "IW{2,1}(248,:)'"/1 -> dotprod248/1
  dotprod248/1 -> Mux/248
  "IW{2,1}(249,:)'"/1 -> dotprod249/1
  dotprod249/1 -> Mux/249
  "IW{2,1}(250,:)'"/1 -> dotprod250/1
  dotprod250/1 -> Mux/250
  "IW{2,1}(251,:)'"/1 -> dotprod251/1
  dotprod251/1 -> Mux/251
  "IW{2,1}(252,:)'"/1 -> dotprod252/1
  dotprod252/1 -> Mux/252
  "IW{2,1}(253,:)'"/1 -> dotprod253/1
  dotprod253/1 -> Mux/253
  "IW{2,1}(254,:)'"/1 -> dotprod254/1
  dotprod254/1 -> Mux/254
  "IW{2,1}(255,:)'"/1 -> dotprod255/1
  dotprod255/1 -> Mux/255
  "IW{2,1}(256,:)'"/1 -> dotprod256/1
  dotprod256/1 -> Mux/256
  "IW{2,1}(257,:)'"/1 -> dotprod257/1
  dotprod257/1 -> Mux/257
  "IW{2,1}(258,:)'"/1 -> dotprod258/1
  dotprod258/1 -> Mux/258
  "IW{2,1}(259,:)'"/1 -> dotprod259/1
  dotprod259/1 -> Mux/259
  "IW{2,1}(260,:)'"/1 -> dotprod260/1
  dotprod260/1 -> Mux/260
  "IW{2,1}(261,:)'"/1 -> dotprod261/1
  dotprod261/1 -> Mux/261
  "IW{2,1}(262,:)'"/1 -> dotprod262/1
  dotprod262/1 -> Mux/262
  "IW{2,1}(263,:)'"/1 -> dotprod263/1
  dotprod263/1 -> Mux/263
  "IW{2,1}(264,:)'"/1 -> dotprod264/1
  dotprod264/1 -> Mux/264
  "IW{2,1}(265,:)'"/1 -> dotprod265/1
  dotprod265/1 -> Mux/265
  "IW{2,1}(266,:)'"/1 -> dotprod266/1
  dotprod266/1 -> Mux/266
  "IW{2,1}(267,:)'"/1 -> dotprod267/1
  dotprod267/1 -> Mux/267
  "IW{2,1}(268,:)'"/1 -> dotprod268/1
  dotprod268/1 -> Mux/268
  "IW{2,1}(269,:)'"/1 -> dotprod269/1
  dotprod269/1 -> Mux/269
  "IW{2,1}(270,:)'"/1 -> dotprod270/1
  dotprod270/1 -> Mux/270
  "IW{2,1}(271,:)'"/1 -> dotprod271/1
  dotprod271/1 -> Mux/271
  "IW{2,1}(272,:)'"/1 -> dotprod272/1
  dotprod272/1 -> Mux/272
  "IW{2,1}(273,:)'"/1 -> dotprod273/1
  dotprod273/1 -> Mux/273
  "IW{2,1}(274,:)'"/1 -> dotprod274/1
  dotprod274/1 -> Mux/274
  "IW{2,1}(275,:)'"/1 -> dotprod275/1
  dotprod275/1 -> Mux/275
  "IW{2,1}(276,:)'"/1 -> dotprod276/1
  dotprod276/1 -> Mux/276
  "IW{2,1}(277,:)'"/1 -> dotprod277/1
  dotprod277/1 -> Mux/277
  "IW{2,1}(278,:)'"/1 -> dotprod278/1
  dotprod278/1 -> Mux/278
  "IW{2,1}(279,:)'"/1 -> dotprod279/1
  dotprod279/1 -> Mux/279
  "IW{2,1}(280,:)'"/1 -> dotprod280/1
  dotprod280/1 -> Mux/280
  "IW{2,1}(281,:)'"/1 -> dotprod281/1
  dotprod281/1 -> Mux/281
  "IW{2,1}(282,:)'"/1 -> dotprod282/1
  dotprod282/1 -> Mux/282
  "IW{2,1}(283,:)'"/1 -> dotprod283/1
  dotprod283/1 -> Mux/283
  "IW{2,1}(284,:)'"/1 -> dotprod284/1
  dotprod284/1 -> Mux/284
  "IW{2,1}(285,:)'"/1 -> dotprod285/1
  dotprod285/1 -> Mux/285
  "IW{2,1}(286,:)'"/1 -> dotprod286/1
  dotprod286/1 -> Mux/286
  "IW{2,1}(287,:)'"/1 -> dotprod287/1
  dotprod287/1 -> Mux/287
  "IW{2,1}(288,:)'"/1 -> dotprod288/1
  dotprod288/1 -> Mux/288
  "IW{2,1}(289,:)'"/1 -> dotprod289/1
  dotprod289/1 -> Mux/289
  "IW{2,1}(290,:)'"/1 -> dotprod290/1
  dotprod290/1 -> Mux/290
  "IW{2,1}(291,:)'"/1 -> dotprod291/1
  dotprod291/1 -> Mux/291
  "IW{2,1}(292,:)'"/1 -> dotprod292/1
  dotprod292/1 -> Mux/292
  "IW{2,1}(293,:)'"/1 -> dotprod293/1
  dotprod293/1 -> Mux/293
  "IW{2,1}(294,:)'"/1 -> dotprod294/1
  dotprod294/1 -> Mux/294
  "IW{2,1}(295,:)'"/1 -> dotprod295/1
  dotprod295/1 -> Mux/295
  "IW{2,1}(296,:)'"/1 -> dotprod296/1
  dotprod296/1 -> Mux/296
  "IW{2,1}(297,:)'"/1 -> dotprod297/1
  dotprod297/1 -> Mux/297
  "IW{2,1}(298,:)'"/1 -> dotprod298/1
  dotprod298/1 -> Mux/298
  "IW{2,1}(299,:)'"/1 -> dotprod299/1
  dotprod299/1 -> Mux/299
  "IW{2,1}(300,:)'"/1 -> dotprod300/1
  dotprod300/1 -> Mux/300
  "IW{2,1}(301,:)'"/1 -> dotprod301/1
  dotprod301/1 -> Mux/301
  "IW{2,1}(302,:)'"/1 -> dotprod302/1
  dotprod302/1 -> Mux/302
  "IW{2,1}(303,:)'"/1 -> dotprod303/1
  dotprod303/1 -> Mux/303
  "IW{2,1}(304,:)'"/1 -> dotprod304/1
  dotprod304/1 -> Mux/304
  "IW{2,1}(305,:)'"/1 -> dotprod305/1
  dotprod305/1 -> Mux/305
  "IW{2,1}(306,:)'"/1 -> dotprod306/1
  dotprod306/1 -> Mux/306
  "IW{2,1}(307,:)'"/1 -> dotprod307/1
  dotprod307/1 -> Mux/307
  "IW{2,1}(308,:)'"/1 -> dotprod308/1
  dotprod308/1 -> Mux/308
  "IW{2,1}(309,:)'"/1 -> dotprod309/1
  dotprod309/1 -> Mux/309
  "IW{2,1}(310,:)'"/1 -> dotprod310/1
  dotprod310/1 -> Mux/310
  "IW{2,1}(311,:)'"/1 -> dotprod311/1
  dotprod311/1 -> Mux/311
  "IW{2,1}(312,:)'"/1 -> dotprod312/1
  dotprod312/1 -> Mux/312
  "IW{2,1}(313,:)'"/1 -> dotprod313/1
  dotprod313/1 -> Mux/313
  "IW{2,1}(314,:)'"/1 -> dotprod314/1
  dotprod314/1 -> Mux/314
  "IW{2,1}(315,:)'"/1 -> dotprod315/1
  dotprod315/1 -> Mux/315
  "IW{2,1}(316,:)'"/1 -> dotprod316/1
  dotprod316/1 -> Mux/316
  "IW{2,1}(317,:)'"/1 -> dotprod317/1
  dotprod317/1 -> Mux/317
  "IW{2,1}(318,:)'"/1 -> dotprod318/1
  dotprod318/1 -> Mux/318
  "IW{2,1}(319,:)'"/1 -> dotprod319/1
  dotprod319/1 -> Mux/319
  "IW{2,1}(320,:)'"/1 -> dotprod320/1
  dotprod320/1 -> Mux/320
  "IW{2,1}(321,:)'"/1 -> dotprod321/1
  dotprod321/1 -> Mux/321
  "IW{2,1}(322,:)'"/1 -> dotprod322/1
  dotprod322/1 -> Mux/322
  "IW{2,1}(323,:)'"/1 -> dotprod323/1
  dotprod323/1 -> Mux/323
  "IW{2,1}(324,:)'"/1 -> dotprod324/1
  dotprod324/1 -> Mux/324
  "IW{2,1}(325,:)'"/1 -> dotprod325/1
  dotprod325/1 -> Mux/325
  "IW{2,1}(326,:)'"/1 -> dotprod326/1
  dotprod326/1 -> Mux/326
  "IW{2,1}(327,:)'"/1 -> dotprod327/1
  dotprod327/1 -> Mux/327
  "IW{2,1}(328,:)'"/1 -> dotprod328/1
  dotprod328/1 -> Mux/328
  "IW{2,1}(329,:)'"/1 -> dotprod329/1
  dotprod329/1 -> Mux/329
  "IW{2,1}(330,:)'"/1 -> dotprod330/1
  dotprod330/1 -> Mux/330
  "IW{2,1}(331,:)'"/1 -> dotprod331/1
  dotprod331/1 -> Mux/331
  "IW{2,1}(332,:)'"/1 -> dotprod332/1
  dotprod332/1 -> Mux/332
  "IW{2,1}(333,:)'"/1 -> dotprod333/1
  dotprod333/1 -> Mux/333
  "IW{2,1}(334,:)'"/1 -> dotprod334/1
  dotprod334/1 -> Mux/334
  "IW{2,1}(335,:)'"/1 -> dotprod335/1
  dotprod335/1 -> Mux/335
  "IW{2,1}(336,:)'"/1 -> dotprod336/1
  dotprod336/1 -> Mux/336
  "IW{2,1}(337,:)'"/1 -> dotprod337/1
  dotprod337/1 -> Mux/337
  "IW{2,1}(338,:)'"/1 -> dotprod338/1
  dotprod338/1 -> Mux/338
  "IW{2,1}(339,:)'"/1 -> dotprod339/1
  dotprod339/1 -> Mux/339
  "IW{2,1}(340,:)'"/1 -> dotprod340/1
  dotprod340/1 -> Mux/340
  "IW{2,1}(341,:)'"/1 -> dotprod341/1
  dotprod341/1 -> Mux/341
  "IW{2,1}(342,:)'"/1 -> dotprod342/1
  dotprod342/1 -> Mux/342
  "IW{2,1}(343,:)'"/1 -> dotprod343/1
  dotprod343/1 -> Mux/343
  "IW{2,1}(344,:)'"/1 -> dotprod344/1
  dotprod344/1 -> Mux/344
  "IW{2,1}(345,:)'"/1 -> dotprod345/1
  dotprod345/1 -> Mux/345
  "IW{2,1}(346,:)'"/1 -> dotprod346/1
  dotprod346/1 -> Mux/346
  "IW{2,1}(347,:)'"/1 -> dotprod347/1
  dotprod347/1 -> Mux/347
  "IW{2,1}(348,:)'"/1 -> dotprod348/1
  dotprod348/1 -> Mux/348
  "IW{2,1}(349,:)'"/1 -> dotprod349/1
  dotprod349/1 -> Mux/349
  "IW{2,1}(350,:)'"/1 -> dotprod350/1
  dotprod350/1 -> Mux/350
  "IW{2,1}(351,:)'"/1 -> dotprod351/1
  dotprod351/1 -> Mux/351
  "IW{2,1}(352,:)'"/1 -> dotprod352/1
  dotprod352/1 -> Mux/352
  "IW{2,1}(353,:)'"/1 -> dotprod353/1
  dotprod353/1 -> Mux/353
  "IW{2,1}(354,:)'"/1 -> dotprod354/1
  dotprod354/1 -> Mux/354
  "IW{2,1}(355,:)'"/1 -> dotprod355/1
  dotprod355/1 -> Mux/355
  "IW{2,1}(356,:)'"/1 -> dotprod356/1
  dotprod356/1 -> Mux/356
  "IW{2,1}(357,:)'"/1 -> dotprod357/1
  dotprod357/1 -> Mux/357
  "IW{2,1}(358,:)'"/1 -> dotprod358/1
  dotprod358/1 -> Mux/358
  "IW{2,1}(359,:)'"/1 -> dotprod359/1
  dotprod359/1 -> Mux/359
  "IW{2,1}(360,:)'"/1 -> dotprod360/1
  dotprod360/1 -> Mux/360
  "IW{2,1}(361,:)'"/1 -> dotprod361/1
  dotprod361/1 -> Mux/361
  "IW{2,1}(362,:)'"/1 -> dotprod362/1
  dotprod362/1 -> Mux/362
  "IW{2,1}(363,:)'"/1 -> dotprod363/1
  dotprod363/1 -> Mux/363
  "IW{2,1}(364,:)'"/1 -> dotprod364/1
  dotprod364/1 -> Mux/364
  "IW{2,1}(365,:)'"/1 -> dotprod365/1
  dotprod365/1 -> Mux/365
  "IW{2,1}(366,:)'"/1 -> dotprod366/1
  dotprod366/1 -> Mux/366
  "IW{2,1}(367,:)'"/1 -> dotprod367/1
  dotprod367/1 -> Mux/367
  "IW{2,1}(368,:)'"/1 -> dotprod368/1
  dotprod368/1 -> Mux/368
  "IW{2,1}(369,:)'"/1 -> dotprod369/1
  dotprod369/1 -> Mux/369
  "IW{2,1}(370,:)'"/1 -> dotprod370/1
  dotprod370/1 -> Mux/370
  "IW{2,1}(371,:)'"/1 -> dotprod371/1
  dotprod371/1 -> Mux/371
  "IW{2,1}(372,:)'"/1 -> dotprod372/1
  dotprod372/1 -> Mux/372
  "IW{2,1}(373,:)'"/1 -> dotprod373/1
  dotprod373/1 -> Mux/373
  "IW{2,1}(374,:)'"/1 -> dotprod374/1
  dotprod374/1 -> Mux/374
  "IW{2,1}(375,:)'"/1 -> dotprod375/1
  dotprod375/1 -> Mux/375
  "IW{2,1}(376,:)'"/1 -> dotprod376/1
  dotprod376/1 -> Mux/376
  "IW{2,1}(377,:)'"/1 -> dotprod377/1
  dotprod377/1 -> Mux/377
  "IW{2,1}(378,:)'"/1 -> dotprod378/1
  dotprod378/1 -> Mux/378
  "IW{2,1}(379,:)'"/1 -> dotprod379/1
  dotprod379/1 -> Mux/379
  "IW{2,1}(380,:)'"/1 -> dotprod380/1
  dotprod380/1 -> Mux/380
  "IW{2,1}(381,:)'"/1 -> dotprod381/1
  dotprod381/1 -> Mux/381
  "IW{2,1}(382,:)'"/1 -> dotprod382/1
  dotprod382/1 -> Mux/382
  "IW{2,1}(383,:)'"/1 -> dotprod383/1
  dotprod383/1 -> Mux/383
  "IW{2,1}(384,:)'"/1 -> dotprod384/1
  dotprod384/1 -> Mux/384
  "IW{2,1}(385,:)'"/1 -> dotprod385/1
  dotprod385/1 -> Mux/385
  "IW{2,1}(386,:)'"/1 -> dotprod386/1
  dotprod386/1 -> Mux/386
  "IW{2,1}(387,:)'"/1 -> dotprod387/1
  dotprod387/1 -> Mux/387
  "IW{2,1}(388,:)'"/1 -> dotprod388/1
  dotprod388/1 -> Mux/388
  "IW{2,1}(389,:)'"/1 -> dotprod389/1
  dotprod389/1 -> Mux/389
  "IW{2,1}(390,:)'"/1 -> dotprod390/1
  dotprod390/1 -> Mux/390
  "IW{2,1}(391,:)'"/1 -> dotprod391/1
  dotprod391/1 -> Mux/391
  "IW{2,1}(392,:)'"/1 -> dotprod392/1
  dotprod392/1 -> Mux/392
  "IW{2,1}(393,:)'"/1 -> dotprod393/1
  dotprod393/1 -> Mux/393
  "IW{2,1}(394,:)'"/1 -> dotprod394/1
  dotprod394/1 -> Mux/394
  "IW{2,1}(395,:)'"/1 -> dotprod395/1
  dotprod395/1 -> Mux/395
  "IW{2,1}(396,:)'"/1 -> dotprod396/1
  dotprod396/1 -> Mux/396
  "IW{2,1}(397,:)'"/1 -> dotprod397/1
  dotprod397/1 -> Mux/397
  "IW{2,1}(398,:)'"/1 -> dotprod398/1
  dotprod398/1 -> Mux/398
  "IW{2,1}(399,:)'"/1 -> dotprod399/1
  dotprod399/1 -> Mux/399
  "IW{2,1}(400,:)'"/1 -> dotprod400/1
  dotprod400/1 -> Mux/400
  "IW{2,1}(401,:)'"/1 -> dotprod401/1
  dotprod401/1 -> Mux/401
  "IW{2,1}(402,:)'"/1 -> dotprod402/1
  dotprod402/1 -> Mux/402
  "IW{2,1}(403,:)'"/1 -> dotprod403/1
  dotprod403/1 -> Mux/403
  "IW{2,1}(404,:)'"/1 -> dotprod404/1
  dotprod404/1 -> Mux/404
  "IW{2,1}(405,:)'"/1 -> dotprod405/1
  dotprod405/1 -> Mux/405
  Mux/1 -> "lz{2,1}"/1
